simulink model "SWC_FDC_type"  (R2021b)
settings: Solver=FixedStepDiscrete  StartTime=0.0  StopTime=10.0  FixedStep=0.001  RelTol=1e-3
values from neighbouring files (symbols this model uses):
  C_TASK_5MS_S = (	C_TICK_TIME_S      	)    [vcu_local_hdr.m]
  DID_VCUKey = uint16(0x0202)    [vcu_local_hdr.m]
  DID_XWD = uint16(513)    [vcu_local_hdr.m]
  DIDLen_DKCKey = uint16(8)    [vcu_local_hdr.m]
  DIDLen_FoxPiBattSta = uint16(4)    [vcu_local_hdr.m]
  DIDLen_FoxPiBrakeSta = uint16(13)    [vcu_local_hdr.m]
  DIDLen_FoxPiButtonSta = uint16(2)    [vcu_local_hdr.m]
  DIDLen_FoxPiCtrlEnSw = uint16(1)    [vcu_local_hdr.m]
  DIDLen_FoxPiDrivingCtrl = uint16(21)    [vcu_local_hdr.m]
  DIDLen_FoxPiEPSSta = uint16(11)    [vcu_local_hdr.m]
  DIDLen_FoxPiLampCtrl = uint16(6)    [vcu_local_hdr.m]
  DIDLen_FoxPiLampSta = uint16(2)    [vcu_local_hdr.m]
  DIDLen_FoxPiMotionSta = uint16(13)    [vcu_local_hdr.m]
  DIDLen_FoxPiMotorSta = uint16(11)    [vcu_local_hdr.m]
  DIDLen_FoxPiPedalPos = uint16(3)    [vcu_local_hdr.m]
  DIDLen_FoxPiPTGUSSSw = uint16(1)    [vcu_local_hdr.m]
  DIDLen_FoxPiShifterAllow = uint16(3)    [vcu_local_hdr.m]
  DIDLen_FoxPiSwSta = uint16(2)    [vcu_local_hdr.m]
  DIDLen_FoxPiTPMSSta = uint16(13)    [vcu_local_hdr.m]
  DIDLen_FoxPiUSSDist = uint16(20)    [vcu_local_hdr.m]
  DIDLen_FoxPiUSSFaultSta = uint16(2)    [vcu_local_hdr.m]
  DIDLen_FoxPiWheelSpd = uint16(16)    [vcu_local_hdr.m]
  DIDNum_DKCKey = uint16(0x0202)    [vcu_local_hdr.m]
  DIDNum_FoxPiBattSta = uint16(0x100D)    [vcu_local_hdr.m]
  DIDNum_FoxPiBrakeSta = uint16(0x1003)    [vcu_local_hdr.m]
  DIDNum_FoxPiButtonSta = uint16(0x1006)    [vcu_local_hdr.m]
  DIDNum_FoxPiCtrlEnSw = uint16(0x1012)    [vcu_local_hdr.m]
  DIDNum_FoxPiDrivingCtrl = uint16(0x1001)    [vcu_local_hdr.m]
  DIDNum_FoxPiEPSSta = uint16(0x1005)    [vcu_local_hdr.m]
  DIDNum_FoxPiLampCtrl = uint16(0x100C)    [vcu_local_hdr.m]
  DIDNum_FoxPiLampSta = uint16(0x100B)    [vcu_local_hdr.m]
  DIDNum_FoxPiMotionSta = uint16(0x1002)    [vcu_local_hdr.m]
  DIDNum_FoxPiMotorSta = uint16(0x1010)    [vcu_local_hdr.m]
  DIDNum_FoxPiPedalPos = uint16(0x100F)    [vcu_local_hdr.m]
  DIDNum_FoxPiPTGUSSSw = uint16(0x1009)    [vcu_local_hdr.m]
  DIDNum_FoxPiShifterAllow = uint16(0x1011)    [vcu_local_hdr.m]
  DIDNum_FoxPiSwSta = uint16(0x100A)    [vcu_local_hdr.m]
  DIDNum_FoxPiTPMSSta = uint16(0x100E)    [vcu_local_hdr.m]
  DIDNum_FoxPiUSSDist = uint16(0x1007)    [vcu_local_hdr.m]
  DIDNum_FoxPiUSSFaultSta = uint16(0x1008)    [vcu_local_hdr.m]
  DIDNum_FoxPiWheelSpd = uint16(0x1004)    [vcu_local_hdr.m]
  DIDVCUKeyLength = uint16(8)    [vcu_local_hdr.m]
  DTC_10020B = Simulink.Parameter    [DTC_Constant_Definition.m]
  DTC_10020C = Simulink.Parameter    [DTC_Constant_Definition.m]
  DTC_10020D = Simulink.Parameter    [DTC_Constant_Definition.m]
  DTC_10020E = Simulink.Parameter    [DTC_Constant_Definition.m]
  DTC_100210 = Simulink.Parameter    [DTC_Constant_Definition.m]
  DTC_100211 = Simulink.Parameter    [DTC_Constant_Definition.m]
  DTC_100212 = Simulink.Parameter    [DTC_Constant_Definition.m]
  DTC_100213 = Simulink.Parameter    [DTC_Constant_Definition.m]
  DTC_100214 = Simulink.Parameter    [DTC_Constant_Definition.m]
  DTC_100215 = Simulink.Parameter    [DTC_Constant_Definition.m]
  DTC_100216 = Simulink.Parameter    [DTC_Constant_Definition.m]
  DTC_100217 = Simulink.Parameter    [DTC_Constant_Definition.m]
  DTC_100218 = Simulink.Parameter    [DTC_Constant_Definition.m]
  DTC_100219 = Simulink.Parameter    [DTC_Constant_Definition.m]
  DTC_10021A = Simulink.Parameter    [DTC_Constant_Definition.m]
  DTC_10021B = Simulink.Parameter    [DTC_Constant_Definition.m]
  DTC_10021C = Simulink.Parameter    [DTC_Constant_Definition.m]
  DTC_10021D = Simulink.Parameter    [DTC_Constant_Definition.m]
  DTC_10021E = Simulink.Parameter    [DTC_Constant_Definition.m]
  DTC_100220 = Simulink.Parameter    [DTC_Constant_Definition.m]
  DTC_100221 = Simulink.Parameter    [DTC_Constant_Definition.m]
  DTC_100223 = Simulink.Parameter    [DTC_Constant_Definition.m]
  DTC_100224 = Simulink.Parameter    [DTC_Constant_Definition.m]
  DTC_100225 = Simulink.Parameter    [DTC_Constant_Definition.m]
  DTC_100226 = Simulink.Parameter    [DTC_Constant_Definition.m]
  DTC_100227 = Simulink.Parameter    [DTC_Constant_Definition.m]
  DTC_100242 = Simulink.Parameter    [DTC_Constant_Definition.m]
  DTC_100243 = Simulink.Parameter    [DTC_Constant_Definition.m]
  DTC_100244 = Simulink.Parameter    [DTC_Constant_Definition.m]
  DTC_100247 = Simulink.Parameter    [DTC_Constant_Definition.m]
  DTC_100248 = Simulink.Parameter    [DTC_Constant_Definition.m]
  DTC_100249 = Simulink.Parameter    [DTC_Constant_Definition.m]
  DTC_100250 = Simulink.Parameter    [DTC_Constant_Definition.m]
  DTC_100251 = Simulink.Parameter    [DTC_Constant_Definition.m]
  DTC_100252 = Simulink.Parameter    [DTC_Constant_Definition.m]
  DTC_100A10 = Simulink.Parameter    [DTC_Constant_Definition.m]
  DTC_100A12 = Simulink.Parameter    [DTC_Constant_Definition.m]
  DTC_100A16 = Simulink.Parameter    [DTC_Constant_Definition.m]
  DTC_100A17 = Simulink.Parameter    [DTC_Constant_Definition.m]
  DTC_100A18 = Simulink.Parameter    [DTC_Constant_Definition.m]
  DTC_100A19 = Simulink.Parameter    [DTC_Constant_Definition.m]
  DTC_500B01 = Simulink.Parameter    [DTC_Constant_Definition.m]
  DTC_500B02 = Simulink.Parameter    [DTC_Constant_Definition.m]
  DTC_500B03 = Simulink.Parameter    [DTC_Constant_Definition.m]
  DTC_500B04 = Simulink.Parameter    [DTC_Constant_Definition.m]
  DTC_500B05 = Simulink.Parameter    [DTC_Constant_Definition.m]
  DTC_500B06 = Simulink.Parameter    [DTC_Constant_Definition.m]
  DTC_500B07 = Simulink.Parameter    [DTC_Constant_Definition.m]
  DTC_500B08 = Simulink.Parameter    [DTC_Constant_Definition.m]
  DTC_500B09 = Simulink.Parameter    [DTC_Constant_Definition.m]
  DTC_500B0A = Simulink.Parameter    [DTC_Constant_Definition.m]
  DTC_500B0B = Simulink.Parameter    [DTC_Constant_Definition.m]
  DTC_500B0C = Simulink.Parameter    [DTC_Constant_Definition.m]
  DTC_500B0D = Simulink.Parameter    [DTC_Constant_Definition.m]
  DTC_500B0E = Simulink.Parameter    [DTC_Constant_Definition.m]
  DTC_500B0F = Simulink.Parameter    [DTC_Constant_Definition.m]
  DTC_500B10 = Simulink.Parameter    [DTC_Constant_Definition.m]
  DTC_90021F = Simulink.Parameter    [DTC_Constant_Definition.m]
  DTC_90022F = Simulink.Parameter    [DTC_Constant_Definition.m]
  DTC_900253 = Simulink.Parameter    [DTC_Constant_Definition.m]
  DTC_900254 = Simulink.Parameter    [DTC_Constant_Definition.m]
  DTC_900301 = Simulink.Parameter    [DTC_Constant_Definition.m]
  DTC_900302 = Simulink.Parameter    [DTC_Constant_Definition.m]
  DTC_900303 = Simulink.Parameter    [DTC_Constant_Definition.m]
  DTC_900304 = Simulink.Parameter    [DTC_Constant_Definition.m]
  DTC_900305 = Simulink.Parameter    [DTC_Constant_Definition.m]
  DTC_900909 = Simulink.Parameter    [DTC_Constant_Definition.m]
  DTC_90090A = Simulink.Parameter    [DTC_Constant_Definition.m]
  DTC_90090B = Simulink.Parameter    [DTC_Constant_Definition.m]
  DTC_90090C = Simulink.Parameter    [DTC_Constant_Definition.m]
  DTC_90090D = Simulink.Parameter    [DTC_Constant_Definition.m]
  DTC_90090E = Simulink.Parameter    [DTC_Constant_Definition.m]
  DTC_90090F = Simulink.Parameter    [DTC_Constant_Definition.m]
  DTC_900910 = Simulink.Parameter    [DTC_Constant_Definition.m]
  DTC_900911 = Simulink.Parameter    [DTC_Constant_Definition.m]
  DTC_900912 = Simulink.Parameter    [DTC_Constant_Definition.m]
  DTC_900913 = Simulink.Parameter    [DTC_Constant_Definition.m]
  DTC_900914 = Simulink.Parameter    [DTC_Constant_Definition.m]
  ... (+54 more)
undefined symbols (not defined in the file or in its folder): f32_ApsOutVehSpdSig, KHAL_CANBusOffDebounce_cnt, KHAL_CANBusOffDebounce_s, KHAL_DKCDecryptEnable_flg_ovrdflg, KHAL_DKCDecryptEnable_flg_ovrdval, KHAL_RandomNumberY1_enum, KHAL_RandomNumberY2_enum, KHAL_RandomNumberY_ovrdflg, KHAL_TPMSRESBUTT_flg_ovrdflg, KHAL_TPMSRESBUTT_flg_ovrdval, KINP_ReadVinCode_flg, P_boolean, R_DIDWriteCDD_CSOP_DIDSet_DKCKey, R_DIDWriteCDD_CSOP_DIDSet_FoxPiBattSta, R_DIDWriteCDD_CSOP_DIDSet_FoxPiBrakeSta, R_DIDWriteCDD_CSOP_DIDSet_FoxPiButtonSta, R_DIDWriteCDD_CSOP_DIDSet_FoxPiCtrlEnSw, R_DIDWriteCDD_CSOP_DIDSet_FoxPiDrivingCtrl, R_DIDWriteCDD_CSOP_DIDSet_FoxPiEPSSta, R_DIDWriteCDD_CSOP_DIDSet_FoxPiLampCtrl, R_DIDWriteCDD_CSOP_DIDSet_FoxPiLampSta, R_DIDWriteCDD_CSOP_DIDSet_FoxPiMotionSta, R_DIDWriteCDD_CSOP_DIDSet_FoxPiMotorSta, R_DIDWriteCDD_CSOP_DIDSet_FoxPiPedalPos, R_DIDWriteCDD_CSOP_DIDSet_FoxPiPTGUSSSw, R_DIDWriteCDD_CSOP_DIDSet_FoxPiShifterAllow, R_DIDWriteCDD_CSOP_DIDSet_FoxPiSwSta, R_DIDWriteCDD_CSOP_DIDSet_FoxPiTPMSSta, R_DIDWriteCDD_CSOP_DIDSet_FoxPiUSSDist, R_DIDWriteCDD_CSOP_DIDSet_FoxPiUSSFaultSta, R_DIDWriteCDD_CSOP_DIDSet_FoxPiWheelSpd, R_E2E_CAN3_VCU1_CSOP_Write_CAN3_VCU1, R_E2E_CAN3_VCU1_toNIDEC_CSOP_Write_CAN3_VCU1_toNIDEC, R_E2E_CAN4_VCU1_CSOP_Write_CAN4_VCU1, R_FDCCDD_Inner_CSOP_FDC_AppCallSleep, R_HALIN_IMU_CSOP_IMUSetSta, R_HALINCDD_CSOP_PAS_Handler, R_HALINCDD_CSOP_ResetPedalZeroPosDone, R_HALINCDD_CSOP_TPMSSensorIDRegSetResults, R_HALINCDD_CSOP_UDS_Main, R_HALOUT_APS_CSOP_ApsOutput, R_HALOUTCDD_CSOP_AppNmStateReq, R_HALOUTCDD_CSOP_IVIReset, R_HALOUTCDD_CSOP_SetAcoreRebootCmdACK, R_HALOUTCDD_CSOP_SetSysPwrStat ... (+80)
libraries: FVT_lib x447, simulink x289, hcu_lib x19, hdlsllib x9, app x1, halin x1, halout x1, matrix_library x1, inp x1, outp x1
(part 3 of 15)

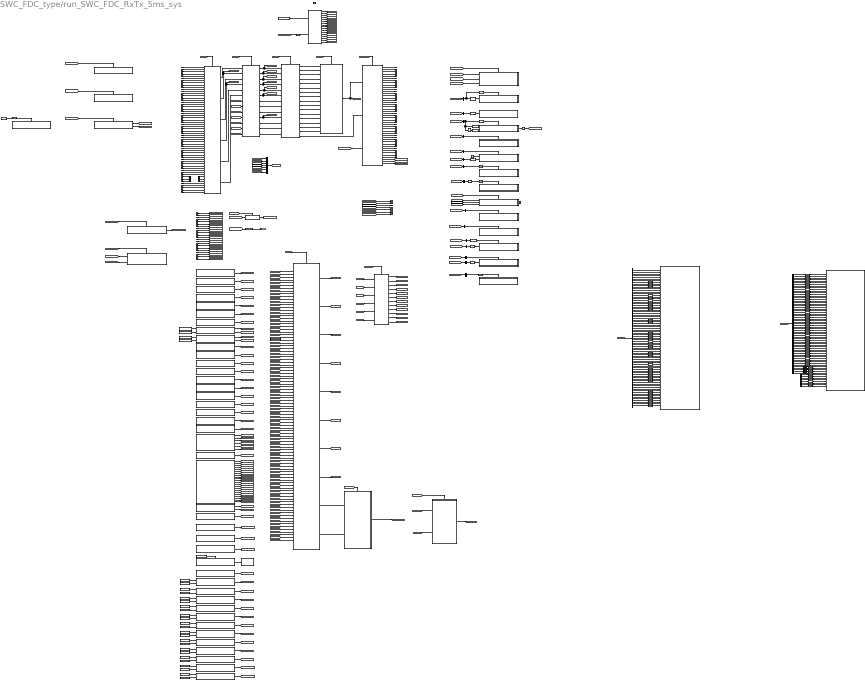
== system SWC_FDC_type/run_SWC_FDC_RxTx_5ms_sys ==
  R_CAN1_ABM1_CAN1_SG_ABM1_read : Inport
  R_CAN1_EPB1_CAN1_SG_EPB1_read : Inport  Port=2
  R_CAN1_EPS1_CAN1_SG_EPS1_read : Inport  Port=3
  R_CAN1_ESC1_CAN1_SG_ESC1_read : Inport  Port=4
  R_CAN1_ESC5_CAN1_SG_ESC5_read : Inport  Port=5
  R_CAN1_eBST1_CAN1_SG_eBST1_read : Inport  Port=6
  R_CAN2_HMI1_CAN2_SG_HMI1_read : Inport  Port=7
  R_CAN2_IVI1_CAN2_SG_IVI1_read : Inport  Port=8
  R_CAN2_IVI2_CAN2_SG_IVI2_read : Inport  Port=9
  R_CAN2_IVI3_CAN2_SG_IVI3_read : Inport  Port=10
  R_CAN2_METER1_CAN2_SG_METER1_read : Inport  Port=11
  R_CAN3_BMS1_CAN3_SG_BMS1_read : Inport  Port=12
  R_CAN3_BMS3_CAN3_SG_BMS3_read : Inport  Port=13
  R_CAN3_BMS4_CAN3_SG_BMS4_read : Inport  Port=14
  R_CAN3_BMS5_CAN3_SG_BMS5_read : Inport  Port=15
  R_CAN3_BMS6_CAN3_SG_BMS6_read : Inport  Port=16
  R_CAN3_BMS8_CAN3_SG_BMS8_read : Inport  Port=17
  R_CAN3_CCU1_CAN3_SG_CCU1_read : Inport  Port=18
  R_CAN3_CCU2_CAN3_SG_CCU2_read : Inport  Port=19
  R_CAN3_EBM1_CAN3_SG_EBM1_read : Inport  Port=20
  R_CAN3_MCU_B_F1_CAN3_SG_MCU_B_F1_read : Inport  Port=21
  R_CAN3_MCU_B_F2_CAN3_SG_MCU_B_F2_read : Inport  Port=22
  R_CAN3_MCU_B_R1_CAN3_SG_MCU_B_R1_read : Inport  Port=23
  R_CAN3_MCU_B_R2_CAN3_SG_MCU_B_R2_read : Inport  Port=24
  R_CAN3_MCU_N_F1_CAN3_SG_MCU_N_F1_read : Inport  Port=25
  R_CAN3_MCU_N_F2_CAN3_SG_MCU_N_F2_read : Inport  Port=26
  R_CAN3_MCU_N_F3_CAN3_SG_MCU_N_F3_read : Inport  Port=27
  R_CAN3_MCU_N_R1_CAN3_SG_MCU_N_R1_read : Inport  Port=28
  R_CAN3_MCU_N_R2_CAN3_SG_MCU_N_R2_read : Inport  Port=29
  R_CAN3_MCU_N_R3_CAN3_SG_MCU_N_R3_read : Inport  Port=30
  R_CAN3_Shifter1_CAN3_SG_Shifter1_read : Inport  Port=31
  R_CAN3_Shifter2_CAN3_SG_Shifter2_read : Inport  Port=32
  R_CAN4_BodyZone_DR1_CAN4_SG_BodyZone_DR1_read : Inport  Port=33
  R_CAN4_BodyZone_PS1_CAN4_SG_BodyZone_PS1_read : Inport  Port=34
  R_CAN4_BodyZone_PS2_CAN4_SG_BodyZone_PS2_read : Inport  Port=35
  R_CAN4_DKC1_CAN4_SG_DKC1_read : Inport  Port=36
  R_CAN4_DKC2_CAN4_SG_DKC2_read : Inport  Port=37
  R_CAN4_PTG1_CAN4_SG_PTG1_read : Inport  Port=38
  R_CAN4_ZONE_DR1_CAN4_SG_ZONE_DR1_read : Inport  Port=39
  R_CAN4_ZONE_DR_VCU_CAN4_SG_ZONE_DR_VCU_read : Inport  Port=40
  R_CAN4_ZONE_FR1_CAN4_SG_ZONE_FR1_read : Inport  Port=41
  R_CAN4_ZONE_FR_VCU_CAN4_SG_ZONE_FR_VCU_read : Inport  Port=42
  R_CAN4_zGW_APTC1_CAN4_SG_zGW_APTC1_read : Inport  Port=43
  R_CAN4_zGW_CANFr1_CAN4_SG_zGW_CANFr1_read : Inport  Port=44
  R_CAN4_zGW_LINDr1_CAN4_SG_zGW_LINDr1_read : Inport  Port=45
  R_CAN4_zGW_LINFr1_CAN4_SG_zGW_LINFr1_read : Inport  Port=46
  R_CAN4_zGW_SEAT1_CAN4_SG_zGW_SEAT1_read : Inport  Port=47
  R_CAN5_TBOX1_CAN5_SG_TBOX1_read : Inport  Port=48
  R_CAN5_TBOX2_CAN5_SG_TBOX2_read : Inport  Port=49
  R_CAN5_TBOX3_CAN5_SG_TBOX3_read : Inport  Port=50
  R_CAN6_FCM1_CAN6_SG_FCM1_read : Inport  Port=51
  R_CAN6_FCM3_CAN6_SG_FCM3_read : Inport  Port=52
  R_CAN6_FCM4_CAN6_SG_FCM4_read : Inport  Port=53
  R_CAN6_SRR1_CAN6_SG_SRR1_read : Inport  Port=54
  IRV_u16Array4_ApsInDist_read : Inport  Port=55
  IRV_u8Array12_ApsInUssSta_read : Inport  Port=56
  IRV_u8Array256_NvmReadArray_read : Inport  Port=57
  IRV_u8Array8_ApsInLevel_read : Inport  Port=58
  IRV_u8Array8_PasInDist_read : Inport  Port=59
  IRV_u8Array9_TPMSData_read : Inport  Port=60
  IRV_u8_ApsInPASChime_read : Inport  Port=61
  IRV_u8_ApsInSensorLayout_read : Inport  Port=62
  IRV_u8_ApsInSysFailSta_read : Inport  Port=63
  IRV_u8_ApsInSysMode_read : Inport  Port=64
  IRV_u8_CTDSW_read : Inport  Port=65
  IRV_u8_CrashSignal_read : Inport  Port=66
  IRV_u8_DrDoorSW_read : Inport  Port=67
  IRV_u8_HazardSW_read : Inport  Port=68
  IRV_u8_HoodSW_read : Inport  Port=69
  IRV_u8_PsDoorSW_read : Inport  Port=70
  IRV_u8_RLDoorSW_read : Inport  Port=71
  IRV_u8_RRDoorSW_read : Inport  Port=72
  IRV_u8_SeatSW_read : Inport  Port=73
  IRV_u8_TPMSDataInSta_read : Inport  Port=74
  IRV_u8_TailgateSW_read : Inport  Port=75
  IRV_u8_TrunkHanSW_read : Inport  Port=76
  R_CAN4_zGW_LINDr2_CAN4_SG_zGW_LINDr2_read : Inport  Port=77
  R_CAN4_zGW_LINFr2_CAN4_SG_zGW_LINFr2_read : Inport  Port=78
  R_CAN6_FCM2_CAN6_SG_FCM2_read : Inport  Port=79
  R_CAN4_BodyZone_DR2_CAN4_SG_BodyZone_DR2_read : Inport  Port=80
  function : TriggerPort  TriggerType=function-call  VariantControl=(inherit)  SampleTimeType=periodic  SampleTime=-1
  APP : app/APP  SystemSampleTime=-1  VariantActivationTime=update diagram  Latency=0  AutoFrameSizeCalculation=off
  Bus Creator : BusCreator  Inputs=7
  Bus Selector : BusSelector  OutputSignals=VOUTP_EnterNewOperCyc_flg
  Bus Selector1 : BusSelector  OutputSignals=VOUTP_AcoreRebootCmdACK_flg
  Bus Selector10 : BusSelector  OutputSignals=VOUTP_NetworkReq_flg
  Bus Selector11 : BusSelector  OutputSignals=VOUTP_SysPowerMode_enum
  Bus Selector12 : BusSelector  OutputSignals=VOUTP_NvWriteReqRisingEdge_flg
  Bus Selector13 : BusSelector  OutputSignals=VOUTP_FdcSlpReqRisingEdge_flg
  Bus Selector14 : BusSelector  OutputSignals=VOUTP_FdcSlpReqRisingEdge_flg
  Bus Selector15 : BusSelector  OutputSignals=VOUTP_FdcSlpReqRisingEdge_flg
  Bus Selector16 : BusSelector  OutputSignals=VOUTP_FdcSlpTime_sec
  Bus Selector17 : BusSelector  OutputSignals=VOUTP_IVIRST_flg
  Bus Selector2 : BusSelector  OutputSignals=VOUTP_IMUEnaCmd_flg
  Bus Selector3 : BusSelector  OutputSignals=VOUTP_PowerSta_enum,VOUTP_BrkPedalPos_pct,VOUTP_ActAPSPosn_pct,VOUTP_LFRawWhlSpeed_kph,VOUTP_RFRawWhlSpeed_kph,VOUTP_LRRawWhlSpeed_kph,VOUTP_RRRawWhlSpeed_kph,VOUTP_LFRawWhlSpeedV_flg,VOUTP_RFRawWhlSpeedV_flg,VOUTP_LRRawWhlSpeedV_flg,VOUTP_RRRawWhlSpeedV_flg,VOUTP_LFWhlRotDir_enum,VOUTP_RFWhlRotDir_enum,VOUTP_LRWhlRotDir_enum,VOUTP_RRWhlRotDir_enum,VOUTP_LFPulseCountV_flg,VOUTP_RFPulseCountV_flg,VOUTP_LRPulseCountV_flg,VOUTP_RRPulseCountV_flg,VOUTP_LFPulseCount_enum,VOUTP_RFPulseCount_enum,VOUTP_LRPulseCount_enum,VOUTP_RRPulseCount_enum,VOUTP_APSActive_flg,VOUTP_APSCtrlAvail_flg,VOUTP_ShifterHandleCmd_enum,VOUTP_DriIntend_enum,VOUTP_EPSAOIControl_enum,VOUTP_SASAngle_Deg,VOUTP_SASSpeed_degps,VOUTP_SASSpeedValid_flg,VOUTP_SASCAL_flg,VOUTP_SASV_flg,VOUTP_GRADE_Deg,VOUTP_YawRate_degps,VOUTP_LatAccel_Gps,VOUTP_LongAccel_Gps,VOUTP_MCPressure_bar,VOUTP_YawRateV_flg,VOUTP_LatAccelV_flg,VOUTP_LongAccelV_flg,VOUTP_MCPressureV_bar,VOUTP_BrkSwSta_flg,VOUTP_BrkSwV_flg,VOUTP_ESCStandstill_flg,VOUTP_ESCAPSSta_enum,VOUTP_EPBExtReleaseAvail_flg,VOUTP_EPBExtApplyAvail_flg,VOUTP_EPBErrSta_enum,VOUTP_EPBSta_enum,VOUTP_AllDoorSW_flg,VOUTP_HoodSW_flg,VOUTP_TailgateSW_flg,VOUTP_AVMparkingcancel_enum,VOUTP_AVMparkingexcute_enum,VOUTP_AVMParkingmode_enum,VOUTP_AVMErrSTA_flg,VOUTP_IVIStatus_flg,VOUTP_CAASSw_enum,VOUTP_IVIScreen_enum,VOUTP_CAASCtrlAvail_flg,VOUTP_ABSActive_flg,VOUTP_TCSActive_flg,VOUTP_DriverSeatBeltCmd_flg,VOUTP_DrDoorSW_flg,VOUTP_PsDoorSW_flg,VOUTP_RLDoorSW_flg,VOUTP_RRDoorSW_flg,VOUTP_RFPressIndi_enum,VOUTP_LFPressIndi_enum,VOUTP_RRPressIndi_enum,VOUTP_LRPressIndi_enum,VOUTP_sigAmbAirT_C,VOUTP_VehActSpd_kph,VOUTP_CAASActive_flg,VOUTP_PwrReqRAPSAvail_flg,VOUTP_DKCPDkeyAreaRAPSSta_enum,VOUTP_DKCParkingModeCmd_enum,VOUTP_PUIDLowPower_flg,VOUTP_DrSeatSta_enum,VOUTP_VCURAPSErrLv2_flg,VOUTP_VCURAPSErrLv3_flg,VOUTP_IVIUserTakeOverAPSSta_flg
  Bus Selector4 : BusSelector  OutputSignals=VOUTP_BrkPedalPosTimeOut_flg,VOUTP_LFRawWhlSpeedTimeOut_flg,VOUTP_RFRawWhlSpeedTimeOut_flg,VOUTP_LRRawWhlSpeedTimeOut_flg,VOUTP_RRRawWhlSpeedTimeOut_flg,VOUTP_LFRawWhlSpeedVTimeOut_flg,VOUTP_RFRawWhlSpeedVTimeOut_flg,VOUTP_LRRawWhlSpeedVTimeOut_flg,VOUTP_RRRawWhlSpeedVTimeOut_flg,VOUTP_LFWhlRotDirTimeOut_flg,VOUTP_RFWhlRotDirTimeOut_flg,VOUTP_LRWhlRotDirTimeOut_flg,VOUTP_RRWhlRotDirTimeOut_flg,VOUTP_LFPulseCountVTimeOut_flg,VOUTP_RFPulseCountVTimeOut_flg,VOUTP_LRPulseCountVTimeOut_flg,VOUTP_RRPulseCountVTimeOut_flg,VOUTP_LFPulseCountTimeOut_flg,VOUTP_RFPulseCountTimeOut_flg,VOUTP_LRPulseCountTimeOut_flg,VOUTP_RRPulseCountTimeOut_flg,VOUTP_ShifterHandleCmdTimeOut_flg,VOUTP_DriIntendTimeOut_flg,VOUTP_EPSAOIControlTimeOut_flg,VOUTP_SASAngleTimeOut_flg,VOUTP_SASSpeedTimeOut_flg,VOUTP_SASSpeedValidTimeOut_flg,VOUTP_SASCALTimeOut_flg,VOUTP_SASVTimeOut_flg,VOUTP_GRADETimeOut_flg,VOUTP_YawRateTimeOut_flg,VOUTP_LatAccelTimeOut_flg,VOUTP_LongAccelTimeOut_flg,VOUTP_MCPressureTimeOut_flg,VOUTP_YawRateVTimeOut_flg,VOUTP_LatAccelVTimeOut_flg,VOUTP_LongAccelVTimeOut_flg,VOUTP_MCPressureVTimeOut_flg,VOUTP_BrkSwStaTimeOut_flg,VOUTP_BrkSwVTimeOut_flg,VOUTP_ESCStandstillTimeOut_flg,VOUTP_ESCAPSStaTimeOut_flg,VOUTP_EPBExtReleaseAvailTimeOut_flg,VOUTP_EPBExtApplyAvailTimeOut_flg,VOUTP_EPBErrStaTimeOut_flg,VOUTP_EPBStaTimeOut_flg,VOUTP_AVMparkingcancelTimeOut_flg,VOUTP_AVMparkingexcuteTimeOut_flg,VOUTP_AVMParkingmodeTimeOut_flg,VOUTP_AVMErrSTATimeOut_flg,VOUTP_IVIStatusTimeOut_flg,VOUTP_CAASSwTimeOut_flg,VOUTP_IVIScreenTimeOut_flg,VOUTP_ABSActiveTimeOut_flg,VOUTP_TCSActiveTimeOut_flg,VOUTP_DriverSeatBeltCmdTimeOut_flg,VOUTP_RFPressIndi_enum,VOUTP_LFPressIndi_enum,VOUTP_RRPressIndi_enum,VOUTP_LRPressIndi_enum,VOUTP_sigAmbAirT_C
  Bus Selector5 : BusSelector  OutputSignals=VOUTP_IMUEnaCmd_flg
  Bus Selector6 : BusSelector  OutputSignals=VHAL_TPMSSensorIDRegResults_raw8
  Bus Selector7 : BusSelector  OutputSignals=VOUTP_TPMSSensorIDRegStart_flg
  Bus Selector8 : BusSelector  OutputSignals=VOUTP_ResetPedalZeroPosStart_flg
  Constant : Constant  Value=DIDVCUKeyLength
  Constant1 : Constant  Value=DID_VCUKey
  Constant{7,10,16..17,21,25,29} (7 alike) : Constant  Value=ZERO_INT
  Constant{6,9,11..13,20,24,28,32} (9 alike) : Constant  Value=ONE_INT
  Constant14 : Constant  Value=TWO_INT
  Constant15 : Constant  Value=TWO_INT
  Constant18 : Constant  Value=THREE_INT
  Constant19 : Constant  Value=THREE_INT
  Constant2 : Constant  Value=uint16(ONE_INT)
  Constant22 : Constant  Value=FOUR_INT
  Constant23 : Constant  Value=FOUR_INT
  Constant26 : Constant  Value=FIVE_INT
  Constant27 : Constant  Value=FIVE_INT
  Constant3 : Constant  Value=DID_XWD
  Constant30 : Constant  Value=SIX_INT
  Constant31 : Constant  Value=SIX_INT
  Constant4 : Constant  Value=TRUE
  Constant5 : Constant  Value=FALSE
  Constant8 : Constant  Value=KINP_ReadVinCode_flg
  DIDGet_Subsystem : Subsystem
  DIDSet_Subsystem : Subsystem
  Data Type Conversion{,1..3,5..13,17..19,21..95,97..107,109..125} (119 alike) : DataTypeConversion  OutDataTypeStr=uint8
  Data Type Conversion{14..16,20} (4 alike) : DataTypeConversion  OutDataTypeStr=int16
  Data Type Conversion4 : DataTypeConversion  OutDataTypeStr=uint32
  Data Type Conversion96 : DataTypeConversion  OutDataTypeStr=single
  Detect Increase : simulink/Logic and Bit Operations/Detect Increase  vinit=0.0  OutDataTypeStr=boolean
  Detect Increase1 : simulink/Logic and Bit Operations/Detect Increase  vinit=0.0  OutDataTypeStr=boolean
  Display : Display
  Function-Call Subsystem : Subsystem  TreatAsAtomicUnit=on
  Ground{,1..8} (9 alike) : Ground
  Ground_{18..24,26} (8 alike) : Ground
  HALOUT_AFTER : Subsystem
  HAL_IN : halin/HAL_IN  SystemSampleTime=-1  VariantActivationTime=update diagram  Latency=0  AutoFrameSizeCalculation=off
  HAL_OUT : halout/HAL_OUT  SystemSampleTime=-1  VariantActivationTime=update diagram  Latency=0  AutoFrameSizeCalculation=off
  Halin_CDD : Subsystem
      settings: RTWSystemCode=Nonreusable function  RTWFcnNameOpts=Use subsystem name  RTWFileNameOpts=Use subsystem name
  INP : inp/INP  SystemSampleTime=-1  VariantActivationTime=update diagram  Latency=0  AutoFrameSizeCalculation=off
  Latch : hcu_lib/Basic_Blocks/Latch
  NOT : Logic  Operator=NOT  Inputs=1  AllPortsSameDT=off  OutDataTypeStr=boolean
  OUTP : outp/OUTP  SystemSampleTime=-1  VariantActivationTime=update diagram  Latency=0  AutoFrameSizeCalculation=off
  OUTP_AFTER : Subsystem
      settings: RTWSystemCode=Nonreusable function  RTWFcnNameOpts=Use subsystem name  RTWFileNameOpts=Use subsystem name
  R_FDCCDD_Inner_CSOP_FDC_AppCallSleep : Subsystem
  R_HALINCDD_CSOP_AnyNmID : FunctionCaller  FunctionPrototype=u8_AnyNMID = R_HALINCDD_CSOP_AnyNmID()  OutputArgumentSpecifications=uint8(1)
  R_HALINCDD_CSOP_CAN1BusOff : FunctionCaller  FunctionPrototype=u8_CAN1BusOff = R_HALINCDD_CSOP_CAN1BusOff()  OutputArgumentSpecifications=uint8(1)
  R_HALINCDD_CSOP_CAN2BusOff : FunctionCaller  FunctionPrototype=u8_CAN2BusOff = R_HALINCDD_CSOP_CAN2BusOff()  OutputArgumentSpecifications=uint8(1)
  R_HALINCDD_CSOP_CAN3BusOff : FunctionCaller  FunctionPrototype=u8_CAN3BusOff = R_HALINCDD_CSOP_CAN3BusOff()  OutputArgumentSpecifications=uint8(1)
  R_HALINCDD_CSOP_CAN4BusOff : FunctionCaller  FunctionPrototype=u8_CAN4BusOff = R_HALINCDD_CSOP_CAN4BusOff()  OutputArgumentSpecifications=uint8(1)
  R_HALINCDD_CSOP_CAN5BusOff : FunctionCaller  FunctionPrototype=u8_CAN5BusOff = R_HALINCDD_CSOP_CAN5BusOff()  OutputArgumentSpecifications=uint8(1)
  R_HALINCDD_CSOP_CAN6BusOff : FunctionCaller  FunctionPrototype=u8_CAN6BusOff = R_HALINCDD_CSOP_CAN6BusOff()  OutputArgumentSpecifications=uint8(1)
  R_HALINCDD_CSOP_DIDgetDKCdata : FunctionCaller  FunctionPrototype=[u8_DidStaDKC,u8Array8_DidDataDKC] = R_HALINCDD_CSOP_DIDgetDKCdata(u16_lengthDIDDKC,u16_DIDDKC)  InputArgumentSpecifications=uint16(1), uint16(1)  OutputArgumentSpecifications=uint8(1), uint8([1;1;1;1;1;1;1;1])
  R_HALINCDD_CSOP_DIDgetXWDdata : FunctionCaller  FunctionPrototype=[u8_DidStaXWD,u8_DidDataXWD] = R_HALINCDD_CSOP_DIDgetXWDdata(u16_lengthDIDXWD,u16_DIDXWD)  InputArgumentSpecifications=uint16(1), uint16(1)  OutputArgumentSpecifications=uint8(1), uint8(1)
  R_HALINCDD_CSOP_GetAcoreReadyToSleep : FunctionCaller  FunctionPrototype=s8_AcoreReadyToSleep = R_HALINCDD_CSOP_GetAcoreReadyToSleep()  OutputArgumentSpecifications=int8(1)
  R_HALINCDD_CSOP_GetAcoreRebootCmd : FunctionCaller  FunctionPrototype=u8_AcoreRebootCmd = R_HALINCDD_CSOP_GetAcoreRebootCmd()  OutputArgumentSpecifications=uint8(1)
  R_HALINCDD_CSOP_GetAuxBattVoltage : FunctionCaller  FunctionPrototype=u16_AuxBattVol100mV = R_HALINCDD_CSOP_GetAuxBattVoltage()  OutputArgumentSpecifications=uint16(1)
  R_HALINCDD_CSOP_GetBootPath : FunctionCaller  FunctionPrototype=u32_BootPath = R_HALINCDD_CSOP_GetBootPath()  OutputArgumentSpecifications=uint32(1)
  R_HALINCDD_CSOP_GetBootReason : FunctionCaller  FunctionPrototype=u8_BootReason = R_HALINCDD_CSOP_GetBootReason()  OutputArgumentSpecifications=uint8(1)
  R_HALINCDD_CSOP_GetEvccAplusPwrUpReq : FunctionCaller  FunctionPrototype=u8_EvccAplusPwrUpReq = R_HALINCDD_CSOP_GetEvccAplusPwrUpReq()  OutputArgumentSpecifications=uint8(1)
  R_HALINCDD_CSOP_GetNmState : FunctionCaller  FunctionPrototype=u8_CurrentNMState = R_HALINCDD_CSOP_GetNmState()  OutputArgumentSpecifications=uint8(1)
  R_HALINCDD_CSOP_GetNvmProtectState : FunctionCaller  FunctionPrototype=u8_NvmProtectSta = R_HALINCDD_CSOP_GetNvmProtectState()  OutputArgumentSpecifications=uint8(1)
  R_HALINCDD_CSOP_GetSWID : FunctionCaller  FunctionPrototype=u8Array33_SWID = R_HALINCDD_CSOP_GetSWID()  OutputArgumentSpecifications=uint8([1;1;1;1;1;1;1;1;1;1;1;1;1;1;1;1;1;1;1;1;1;1;1;1;1;1;1;1;1;1;1;1;1])
  R_HALINCDD_CSOP_GetVinpAllowMoveThdOta : FunctionCaller  FunctionPrototype=u8_AllowMovThdOTA = R_HALINCDD_CSOP_GetVinpAllowMoveThdOta()  OutputArgumentSpecifications=uint8(1)
  R_HALINCDD_CSOP_GetVinpPwrReqOta : FunctionCaller  FunctionPrototype=u8_PwrReqOTA = R_HALINCDD_CSOP_GetVinpPwrReqOta()  OutputArgumentSpecifications=uint8(1)
  R_HALINCDD_CSOP_GetWISR : FunctionCaller  FunctionPrototype=u32_WISR = R_HALINCDD_CSOP_GetWISR()  OutputArgumentSpecifications=uint32(1)
  R_HALINCDD_CSOP_HALINCDD_DIRECT : FunctionCaller  FunctionPrototype=[u8_BrakeSW,u8_BrakeLamp,u16_Pedal1Vol,u16_Pedal2Vol,u16_Pedal1Ref5V,u16_Pedal2Ref5V] = R_HALINCDD_CSOP_HALINCDD_DIRECT()  OutputArgumentSpecifications=uint8(1), uint8(1), uint16(1), uint16(1), uint16(1), uint16(1)
  R_HALINCDD_CSOP_ReadPedalZeroPosReq : FunctionCaller  FunctionPrototype=u8_ReadPedalZeroPosReq = R_HALINCDD_CSOP_ReadPedalZeroPosReq()  OutputArgumentSpecifications=uint8(1)
  R_HALINCDD_CSOP_ResetPedalZeroPosReq : FunctionCaller  FunctionPrototype=u8_ResetPedalZeroPosReq = R_HALINCDD_CSOP_ResetPedalZeroPosReq()  OutputArgumentSpecifications=uint8(1)
  R_HALINCDD_CSOP_TPMSSensorIDRegGetSta : FunctionCaller  FunctionPrototype=u8_TPMSSensorIDRegSta = R_HALINCDD_CSOP_TPMSSensorIDRegGetSta()  OutputArgumentSpecifications=uint8(1)
  R_HALINCDD_CSOP_nmGetCan1RxErrorCount : FunctionCaller  FunctionPrototype=u8_pCan1RxErrorCount = R_HALINCDD_CSOP_nmGetCan1RxErrorCount(u8_canChannel,u8_isGetRx)  InputArgumentSpecifications=uint8(1), uint8(1)  OutputArgumentSpecifications=uint8(1)
  R_HALINCDD_CSOP_nmGetCan1TxErrorCount : FunctionCaller  FunctionPrototype=u8_pCan1TxErrorCount = R_HALINCDD_CSOP_nmGetCan1TxErrorCount(u8_canChannel,u8_isGetRx)  InputArgumentSpecifications=uint8(1), uint8(1)  OutputArgumentSpecifications=uint8(1)
  R_HALINCDD_CSOP_nmGetCan2RxErrorCount : FunctionCaller  FunctionPrototype=u8_pCan2RxErrorCount = R_HALINCDD_CSOP_nmGetCan2RxErrorCount(u8_canChannel,u8_isGetRx)  InputArgumentSpecifications=uint8(1), uint8(1)  OutputArgumentSpecifications=uint8(1)
  R_HALINCDD_CSOP_nmGetCan2TxErrorCount : FunctionCaller  FunctionPrototype=u8_pCan2TxErrorCount = R_HALINCDD_CSOP_nmGetCan2TxErrorCount(u8_canChannel,u8_isGetRx)  InputArgumentSpecifications=uint8(1), uint8(1)  OutputArgumentSpecifications=uint8(1)
  R_HALINCDD_CSOP_nmGetCan3RxErrorCount : FunctionCaller  FunctionPrototype=u8_pCan3RxErrorCount = R_HALINCDD_CSOP_nmGetCan3RxErrorCount(u8_canChannel,u8_isGetRx)  InputArgumentSpecifications=uint8(1), uint8(1)  OutputArgumentSpecifications=uint8(1)
  R_HALINCDD_CSOP_nmGetCan3TxErrorCount : FunctionCaller  FunctionPrototype=u8_pCan3TxErrorCount = R_HALINCDD_CSOP_nmGetCan3TxErrorCount(u8_canChannel,u8_isGetRx)  InputArgumentSpecifications=uint8(1), uint8(1)  OutputArgumentSpecifications=uint8(1)
  R_HALINCDD_CSOP_nmGetCan4RxErrorCount : FunctionCaller  FunctionPrototype=u8_pCan4RxErrorCount = R_HALINCDD_CSOP_nmGetCan4RxErrorCount(u8_canChannel,u8_isGetRx)  InputArgumentSpecifications=uint8(1), uint8(1)  OutputArgumentSpecifications=uint8(1)
  R_HALINCDD_CSOP_nmGetCan4TxErrorCount : FunctionCaller  FunctionPrototype=u8_pCan4TxErrorCount = R_HALINCDD_CSOP_nmGetCan4TxErrorCount(u8_canChannel,u8_isGetRx)  InputArgumentSpecifications=uint8(1), uint8(1)  OutputArgumentSpecifications=uint8(1)
  R_HALINCDD_CSOP_nmGetCan5RxErrorCount : FunctionCaller  FunctionPrototype=u8_pCan5RxErrorCount = R_HALINCDD_CSOP_nmGetCan5RxErrorCount(u8_canChannel,u8_isGetRx)  InputArgumentSpecifications=uint8(1), uint8(1)  OutputArgumentSpecifications=uint8(1)
  R_HALINCDD_CSOP_nmGetCan5TxErrorCount : FunctionCaller  FunctionPrototype=u8_pCan5TxErrorCount = R_HALINCDD_CSOP_nmGetCan5TxErrorCount(u8_canChannel,u8_isGetRx)  InputArgumentSpecifications=uint8(1), uint8(1)  OutputArgumentSpecifications=uint8(1)
  R_HALINCDD_CSOP_nmGetCan6RxErrorCount : FunctionCaller  FunctionPrototype=u8_pCan6RxErrorCount = R_HALINCDD_CSOP_nmGetCan6RxErrorCount(u8_canChannel,u8_isGetRx)  InputArgumentSpecifications=uint8(1), uint8(1)  OutputArgumentSpecifications=uint8(1)
  R_HALINCDD_CSOP_nmGetCan6TxErrorCount : FunctionCaller  FunctionPrototype=u8_pCan6TxErrorCount = R_HALINCDD_CSOP_nmGetCan6TxErrorCount(u8_canChannel,u8_isGetRx)  InputArgumentSpecifications=uint8(1), uint8(1)  OutputArgumentSpecifications=uint8(1)
  R_HALINCDD_u8Array4_HWID : FunctionCaller  FunctionPrototype=u8Array4_HWID = R_HALINCDD_u8Array4_HWID()  OutputArgumentSpecifications=uint8([1;1;1;1])
  R_HALIN_APS_CSOP_ApsGetData : FunctionCaller  FunctionPrototype=[u8_GetAPS_Progress_PCT,u8_GetAPS_RQ_Display,u8_GetAPS_SW_Ver,u8_GetAPS_HW_Ver,u8_GetAPS_ExitCondition,f32_GetAPS_Angle_Target,u8_GetAPS_Sta_System,u8_GetAPS_V_Rq_EPAS_Ctrl,u8_GetAPS_Rq_EPAS_Ctrl,u8_GetAPS_Req,f32_GetAPS_DecReq,u8_GetAPS_DecReq_A,f32_GetAPS_SpeedCmd,u8_GetAPS_ShftPosnReq,u8_GetAPS_VMC_Req_A,u8_GetCAAS_Sta,u8_GetCAAS_VMC_Req_A,u8_GetAPS_PwrReq_cmd,u8_GetRAPS_BCM_LockReq_Cmd,u8_GetRAPS_BCM_Lamp_Cmd,u8_GetRAPS_ErrWarn_Sta,u8_GetRAPS_ErrLv1_flg] = R_HALIN_APS_CSOP_ApsGetData()  OutputArgumentSpecifications=uint8(1), uint8(1), uint8(1), uint8(1), uint8(1), single(1), uint8(1), uint8(1), uint8(1), uint8(1), single(1), uint8(1), single(1), uint8(1), uint8(1), uint8(1), uint8(1), uint8(1), uint8(1), uint8(1), uint8(1), uint8(1)
  R_HALIN_IMU_CSOP_IMUGetOffsetVal : Subsystem
  R_HALIN_IMU_CSOP_IMUGetSixAxisVal : FunctionCaller  FunctionPrototype=[s16_IMUSixAxisVal,u8_IMUSixAxisValSta] = R_HALIN_IMU_CSOP_IMUGetSixAxisVal()  OutputArgumentSpecifications=int16([1;1;1;1;1;1]), uint8(1)
  R_HALIN_IMU_CSOP_IMUSetSta : Subsystem
  R_HALOUTCDD_CSOP_AppNmStateReq : Subsystem
  R_HALOUTCDD_CSOP_SetAcoreRebootCmdACK : Subsystem
  R_HALOUTCDD_CSOP_SetSysPwrStat : FunctionCaller  FunctionPrototype=R_HALOUTCDD_CSOP_SetSysPwrStat(u8_SysPwrStat)  InputArgumentSpecifications=uint8(1)
  R_HALOUTCDD_CSOP_SleepRequest : Subsystem
  R_HALOUT_APS_CSOP_ApsSetData : FunctionCaller  FunctionPrototype=R_HALOUT_APS_CSOP_ApsSetData(u8_SetPwrSta,f32_SetBrkPedalPos,f32_SetActAPSPosn,f32_SetLF_RawWhlSpeed,f32_SetRF_RawWhlSpeed,f32_SetLR_RawWhlSpeed,f32_SetRR_RawWhlSpeed,u8_SetLF_RawWhlSpeed_V,u8_SetRF_RawWhlSpeed_V,u8_SetLR_RawWhlSpeed_V,u8_SetRR_RawWhlSpeed_V,u8_SetLF_WhlRotDir,u8_SetRF_WhlRotDir,u8_SetLR_WhlRotDir,u8_SetRR_WhlRotDir,u8_SetLF_PulseCount_V,u8_SetRF_PulseCount_V,u8_SetLR_PulseCount_V,u8_SetRR_PulseCount_V,s16_SetLF_PulseCount,s16_SetRF_PulseCount,s16_SetLR_PulseCount,s16_SetRR_PulseCount,u8_SetAPS_Active,u8_SetAPS_CtrlAvail,u8_SetShifter_Handle_Cmd,u8_SetDriIntend,u8_SetEPS_AOI_Control,f32_SetSAS_Angle,f32_SetSAS_Speed,u8_SetSAS_Speed_Valid,u8_SetSAS_CAL,u8_SetSAS_OK,f32_SetGRADE,f32_SetYawRate,f32_SetLatAccel,f32_SetLongAccel,f32_SetMCPressure,u8_SetYawRate_V,u8_SetLatAccel_V,u8_SetLongAccel_V,u8_SetMCPressure_V,u8_SetBrkSw_Sta,u8_SetBrkSw_V,u8_SetESC_Standstill,u8_SetESC_APS_Sta,u8_SetEPBExtReleaseAvail,u8_SetEPBExtApplyAvail,u8_SetEPBErrSta,u8_SetEPBSta,u8_SetAllDoorSW,u8_SetHoodSW,u8_SetTailgate_SW,u8_SetAVM_parking_cancel,u8_SetAVM_parking_excute,u8_SetAVM_Parking_mode,u8_SetAVM_Err_STA,u8_SetIVI_Status,u8_SetCAAS_Sw,u8_SetIVI_Screen,u8_SetCAAS_CtrlAvail,u8_SetABS_Active,u8_SetTCS_Active,u8_SetDriverSeatBeltCmd,u8_SetDrDoorSW,u8_SetPsDoorSW,u8_SetRLDoorSW,u8_SetRRDoorSW,u8_SetRFPressIndi,u8_SetLFPressIndi,u8_SetRRPressIndi,u8_SetLRPressIndi,f32_SetsigAmbAirT,f32_SetVehActSpd,u8_SetCAAS_Active,u8_SetAPS_PwrReqAvail_sta,u8_SetDKC_PDkeyAreaRAPS_Sta,u8_SetDKC_ParkingMode_Cmd,u8_SetP_UID_LowPower,u8_SetDr_SeatSta,u8_SetVCU_RAPSErrLv2_flg,u8_SetVCU_RAPSErrLv3_flg,u8_SetIVI_UserTakeOver_APS_Sta)  InputArgumentSpecifications=uint8(1), single(1), single(1), single(1), single(1), single(1), single(1), uint8(1), uint8(1), uint8(1), uint8(1), uint8(1), uint8(1), uint8(1), uint8(1), uint8(1), uint8(1), uint8(1), uint8(1), int16(1), int16(1), int16(1), int16(1), uint8(1), uint8(1), uint8(1), uint8(1), uint8(1), single(1), single(1), uint8(1), uint8(1), uint8(1), single(1), single(1), single(1), single(1), single(1), uint8(1), uint8(1), uint8(1), uint8(1), uint8(1), uint8(1), uint8(1), uint8(1), uint8(1), uint8(1), uint8(1), uint8(1), uint8(1), uint8(1), uint8(1), uint8(1), uint8(1), uint8(1), uint8(1), uint8(1), uint8(1), uint8(1), uint8(1), uint8(1), uint8(1), uint8(1), uint8(1), uint8(1), uint8(1), uint8(1), uint8(1), uint8(1), uint8(1), uint8(1), single(1), single(1), uint8(1), uint8(1), uint8(1), uint8(1), uint8(1), uint8(1), uint8(1), uint8(1), uint8(1)
  R_HALOUT_APS_CSOP_ApsSetTimeout : FunctionCaller  FunctionPrototype=R_HALOUT_APS_CSOP_ApsSetTimeout(u8_SetBrkPedalPosTO,u8_SetLF_RawWhlSpeedTO,u8_SetRF_RawWhlSpeedTO,u8_SetLR_RawWhlSpeedTO,u8_SetRR_RawWhlSpeedTO,u8_SetLF_RawWhlSpeed_VTO,u8_SetRF_RawWhlSpeed_VTO,u8_SetLR_RawWhlSpeed_VTO,u8_SetRR_RawWhlSpeed_VTO,u8_SetLF_WhlRotDirTO,u8_SetRF_WhlRotDirTO,u8_SetLR_WhlRotDirTO,u8_SetRR_WhlRotDirTO,u8_SetLF_PulseCount_VTO,u8_SetRF_PulseCount_VTO,u8_SetLR_PulseCount_VTO,u8_SetRR_PulseCount_VTO,u8_SetLF_PulseCountTO,u8_SetRF_PulseCountTO,u8_SetLR_PulseCountTO,u8_SetRR_PulseCountTO,u8_SetShifter_Handle_CmdTO,u8_SetDriIntendTO,u8_SetEPS_AOI_ControlTO,u8_SetSAS_AngleTO,u8_SetSAS_SpeedTO,u8_SetSAS_Speed_ValidTO,u8_SetSAS_CALTO,u8_SetSAS_OKTO,u8_SetGRADETO,u8_SetYawRateTO,u8_SetLatAccelTO,u8_SetLongAccelTO,u8_SetMCPressureTO,u8_SetYawRate_VTO,u8_SetLatAccel_VTO,u8_SetLongAccel_VTO,u8_SetMCPressure_VTO,u8_SetBrkSw_StaTO,u8_SetBrkSw_VTO,u8_SetESC_StandstillTO,u8_SetESC_APS_StaTO,u8_SetEPBExtReleaseAvailTO,u8_SetEPBExtApplyAvailTO,u8_SetEPBErrStaTO,u8_SetEPBStaTO,u8_SetAVM_parking_cancelTO,u8_SetAVM_parking_excuteTO,u8_SetAVM_Parking_modeTO,u8_SetAVM_Err_STATO,u8_SetIVI_StatusTO,u8_SetCAAS_SwTO,u8_SetIVI_ScreenTO,u8_SetABS_ActiveTO,u8_SetTCS_ActiveTO,u8_SetDriverSeatBeltCmdTO,u8_SetRFPressIndiTO,u8_SetLFPressIndiTO,u8_SetRRPressIndiTO,u8_SetLRPressIndiTO,u8_SetsigAmbAirTTO,u8_SetAPS_PwrReqAvail_staTO,u8_SetDKC_PDkeyAreaRAPS_StaTO,u8_SetDKC_ParkingMode_CmdTO,u8_SetP_UID_LowPowerTO,u8_SetDr_SeatStaTO,u8_SetVCU_RAPSErrLv2_flgTO,u8_SetVCU_RAPSErrLv3_flgTO,u8_SetIVI_UserTakeOver_APS_StaTO)  InputArgumentSpecifications=uint8(1), uint8(1), uint8(1), uint8(1), uint8(1), uint8(1), uint8(1), uint8(1), uint8(1), uint8(1), uint8(1), uint8(1), uint8(1), uint8(1), uint8(1), uint8(1), uint8(1), uint8(1), uint8(1), uint8(1), uint8(1), uint8(1), uint8(1), uint8(1), uint8(1), uint8(1), uint8(1), uint8(1), uint8(1), uint8(1), uint8(1), uint8(1), uint8(1), uint8(1), uint8(1), uint8(1), uint8(1), uint8(1), uint8(1), uint8(1), uint8(1), uint8(1), uint8(1), uint8(1), uint8(1), uint8(1), uint8(1), uint8(1), uint8(1), uint8(1), uint8(1), uint8(1), uint8(1), uint8(1), uint8(1), uint8(1), uint8(1), uint8(1), uint8(1), uint8(1), uint8(1), uint8(1), uint8(1), uint8(1), uint8(1), uint8(1), uint8(1), uint8(1), uint8(1)
  R_NVMReadCDD_Inner_NVM_ReadOperation : Subsystem
  R_NVMWriteCDD_Inner_NVM_WriteOperation : Subsystem
  R_UDSCDD_CSOP_DdmClearDTCNotification : FunctionCaller  FunctionPrototype=u8_ClearDTCcmd = R_UDSCDD_CSOP_DdmClearDTCNotification()  OutputArgumentSpecifications=uint8(1)
  R_UDSCDD_CSOP_DdmRestartOperationCycle : Subsystem
  R_UDSCDD_CSOP_SetDTCStatus : Subsystem
  R_WDGCDD_CSOP_Call_WDG_AppEnd : Subsystem
  R_WDGCDD_CSOP_Call_WDG_AppStart : Subsystem
  R_WDGCDD_CSOP_Call_Watchdog : Subsystem
  Real_DetectChange : hcu_lib/Basic_Blocks/Real_DetectChange
  Subsystem : Subsystem
  Subsystem1 : Subsystem
  Subsystem3 : Subsystem
  Subsystem4 : Subsystem
  Subsystem5 : Subsystem
  Subsystem6 : Subsystem
  Subsystem7 : Subsystem
  Terminator{,1..7} (8 alike) : Terminator
  Terminator_11 : Terminator
  Unit Delay{,1..3} (4 alike) : UnitDelay  SampleTime=-1  HasFrameUpgradeWarning=on
  detect_Increase : simulink/Logic and Bit Operations/Detect Increase  vinit=0.0  OutDataTypeStr=boolean
  detect_change : simulink/Logic and Bit Operations/Detect Change  vinit=0  OutDataTypeStr=boolean
  detect_change1 : simulink/Logic and Bit Operations/Detect Change  vinit=0  OutDataTypeStr=boolean
  hcu_main_sched : Stateflow chart  TreatAsAtomicUnit=on
      settings: PortSchema="{\"entries\":[{\"content\":{\"sides\":[{\"content\":{\"connectorIds\":[\"In1\",\"In2\"]},\"type\":\"ConnectorPlacement.EquallySpacedRectSide\",\"uuid\":\"b7e373d4-7b92-4563-a962-1396bf0d3836\"},{\"content\":{\"connectorIds\":[\"Out1\",\"Out16\",\"Out2\",\"Out3\",\"Out4\",\"Out5\",\"Out6\",\"Out7\",\"Out8\",\"Out9\",\"Out10\",\"Out11\",\"Out12\",\"Out13\",\"Out17\",\"Out14\",\"Out15\"],\"side\":\"RIGHT\"},\"type\":\"ConnectorPlacement.EquallySpacedRectSide\",\"uuid\":\"9162eed8-852f-437e-b7a7-3f514daa5dad\"},{\"content\":{\"connectorIds\":[],\"side\":\"TOP\"},\"type\":\"ConnectorPlacement.EquallySpacedRectSide\",\"uuid\":\"4ba5874d-9ced-4b78-a5b9-28a1ade43d03\"}]},\"type\":\"ConnectorPlacement.EquallySpacedConnector\",\"uuid\":\"986bc96e-cdd1-4540-b0f0-d43c4f1d98ba\"}],\"packageUris\":[\"http://schema.mathworks.com/mf0/Connector/R2020b\"],\"version\":\"1.0\"}"
  P_CAN1_FD1_BCM1_CAN1_SG_FD1_BCM1_write : Outport
  P_CAN1_FD1_VCU1_CAN1_SG_FD1_VCU1_write : Outport  Port=2
  P_CAN1_FD1_VMC1_CAN1_SG_FD1_VMC1_write : Outport  Port=3
  P_CAN2_FD2_CE100_0_CAN2_SG_FD2_CE100_0_write : Outport  Port=4
  P_CAN2_FD2_CE200_1_CAN2_SG_FD2_CE200_1_write : Outport  Port=5
  P_CAN2_GW2_CE100_0_CAN2_SG_GW2_CE100_0_write : Outport  Port=6
  P_CAN2_GW2_CE200_0_CAN2_SG_GW2_CE200_0_write : Outport  Port=7
  P_CAN3_FD3_BCM1_CAN3_SG_FD3_BCM1_write : Outport  Port=8
  P_CAN3_FD3_THCM2_CAN3_SG_FD3_THCM2_write : Outport  Port=9
  P_CAN3_FD3_V2L1_CAN3_SG_FD3_V2L1_write : Outport  Port=10
  P_CAN4_FD4_CE100_1_CAN4_SG_FD4_CE100_1_write : Outport  Port=11
  P_CAN4_FD4_CE200_0_CAN4_SG_FD4_CE200_0_write : Outport  Port=12
  P_CAN4_GW4_CE100_0_CAN4_SG_GW4_CE100_0_write : Outport  Port=13
  P_CAN5_FD5_CE100_0_CAN5_SG_FD5_CE100_0_write : Outport  Port=14
  P_CAN5_FD5_Debug1_CAN5_SG_FD5_Debug1_write : Outport  Port=15
  P_CAN5_FD5_Debug2_CAN5_SG_FD5_Debug2_write : Outport  Port=16
  P_CAN6_FD6_BCM1_CAN6_SG_FD6_BCM1_write : Outport  Port=17
  P_CAN6_FD6_VCU1_CAN6_SG_FD6_VCU1_write : Outport  Port=18
  P_CAN6_FD6_VMC1_CAN6_SG_FD6_VMC1_write : Outport  Port=19
  P_CAN6_GW6_CE100_0_CAN6_SG_GW6_CE100_0_write : Outport  Port=20
  IRV_ms10_CAN1_SG_FD1_APS3_write : Outport  Port=21  OutDataTypeStr=Bus: DT_CAN1_SG_FD1_APS3  PortDimensions=1  BusOutputAsStruct=on
  IRV_ms10_CAN1_SG_FD1_VCU2_write : Outport  Port=22  OutDataTypeStr=Bus: DT_CAN1_SG_FD1_VCU2  PortDimensions=1  BusOutputAsStruct=on
  IRV_ms10_CAN1_SG_FD1_VCU3_write : Outport  Port=23  OutDataTypeStr=Bus: DT_CAN1_SG_FD1_VCU3  PortDimensions=1  BusOutputAsStruct=on
  IRV_ms10_CAN1_SG_VMC_FCM1_write : Outport  Port=24  OutDataTypeStr=Bus: DT_CAN1_SG_VMC_FCM1  PortDimensions=1  BusOutputAsStruct=on
  IRV_ms10_CAN3_SG_FD3_VCU0_write : Outport  Port=25  OutDataTypeStr=Bus: DT_CAN3_SG_FD3_VCU0  PortDimensions=1  BusOutputAsStruct=on
  IRV_ms10_CAN3_SG_FD3_VCU2_write : Outport  Port=26  OutDataTypeStr=Bus: DT_CAN3_SG_FD3_VCU2  PortDimensions=1  BusOutputAsStruct=on
  IRV_ms10_CAN3_SG_FD3_VCU2_toNIDEC_write : Outport  Port=27  OutDataTypeStr=Bus: DT_CAN3_SG_FD3_VCU2_toNIDEC  PortDimensions=1  BusOutputAsStruct=on
  IRV_ms10_CAN3_SG_FD3_VCU5_write : Outport  Port=28  OutDataTypeStr=Bus: DT_CAN3_SG_FD3_VCU5  PortDimensions=1  BusOutputAsStruct=on
  IRV_ms10_CAN3_SG_GW_ESC1_toNIDEC_write : Outport  Port=29  OutDataTypeStr=Bus: DT_CAN3_SG_GW_ESC1_toNIDEC  PortDimensions=1  BusOutputAsStruct=on
  IRV_ms10_CAN5_SG_FD5_Debug3_write : Outport  Port=30  OutDataTypeStr=Bus: DT_CAN5_SG_FD5_Debug3  PortDimensions=1  BusOutputAsStruct=on
  IRV_ms10_CAN6_SG_FD6_APS3_write : Outport  Port=31  OutDataTypeStr=Bus: DT_CAN6_SG_FD6_APS3  PortDimensions=1  BusOutputAsStruct=on
  IRV_ms10_CAN6_SG_FD6_VCU2_write : Outport  Port=32  OutDataTypeStr=Bus: DT_CAN6_SG_FD6_VCU2  PortDimensions=1  BusOutputAsStruct=on
  IRV_ms100_CAN1_SG_FD1_THCM1_write : Outport  Port=33  OutDataTypeStr=Bus: DT_CAN1_SG_FD1_THCM1  PortDimensions=1  BusOutputAsStruct=on
  IRV_ms100_CAN3_SG_FD3_THCM1_write : Outport  Port=34  OutDataTypeStr=Bus: DT_CAN3_SG_FD3_THCM1  PortDimensions=1  BusOutputAsStruct=on
  IRV_ms1000_CAN3_SG_GW_IVI6_toNIDEC_write : Outport  Port=35  OutDataTypeStr=Bus: DT_CAN3_SG_GW_IVI6_toNIDEC  PortDimensions=1  BusOutputAsStruct=on
  IRV_ms20_CAN1_SG_FD1_APS2_write : Outport  Port=36  OutDataTypeStr=Bus: DT_CAN1_SG_FD1_APS2  PortDimensions=1  BusOutputAsStruct=on
  IRV_ms20_CAN2_SG_FD2_C20_0_write : Outport  Port=37  OutDataTypeStr=Bus: DT_CAN2_SG_FD2_C20_0  PortDimensions=1  BusOutputAsStruct=on
  IRV_ms500_CAN1_SG_FD1_VMC2_write : Outport  Port=38  OutDataTypeStr=Bus: DT_CAN1_SG_FD1_VMC2  PortDimensions=1  BusOutputAsStruct=on
  IRV_ms5000_CAN2_SG_FD2_Version_write : Outport  Port=39  OutDataTypeStr=Bus: DT_CAN2_SG_FD2_Version  PortDimensions=1  BusOutputAsStruct=on
  IRV_E2E_CAN3_SG_FD3_VCU1_write : Outport  Port=40  OutDataTypeStr=Bus: DT_CAN3_SG_FD3_VCU1  PortDimensions=1  BusOutputAsStruct=on
  IRV_E2E_CAN3_SG_FD3_VCU1_toNIDEC_write : Outport  Port=41  OutDataTypeStr=Bus: DT_CAN3_SG_FD3_VCU1_toNIDEC  PortDimensions=1  BusOutputAsStruct=on
  IRV_E2E_CAN4_SG_FD4_CE100_0_write : Outport  Port=42  OutDataTypeStr=Bus: DT_CAN4_SG_FD4_CE100_0  PortDimensions=1  BusOutputAsStruct=on
  IRV_f32_ApsOutVehSpdSig_write : Outport  Port=43  OutDataTypeStr=single  PortDimensions=1
  IRV_u8Array256_NvmWriteArray_write : Outport  Port=44  OutDataTypeStr=uint8  PortDimensions=256
  IRV_u8_ApsOutGearPosnSig_write : Outport  Port=45  OutDataTypeStr=uint8  PortDimensions=1
  IRV_u8_ApsOutSendChrgPlugSta_write : Outport  Port=46  OutDataTypeStr=uint8  PortDimensions=1
  IRV_u8_ApsOutSetFrSensorOnCmd_write : Outport  Port=47  OutDataTypeStr=uint8  PortDimensions=1
  IRV_u8_ApsOutSetFrSensorSwTOCmd_write : Outport  Port=48  OutDataTypeStr=uint8  PortDimensions=1
  IRV_u8_ApsOutSetVehSpdTOCmd_write : Outport  Port=49  OutDataTypeStr=uint8  PortDimensions=1
  wires:
  IRV_u16Array4_ApsInDist_read/1 -> [u16Array4_ApsInDist]
  IRV_u8Array12_ApsInUssSta_read/1 -> [u8Array12_ApsInUssSta]
  IRV_u8Array256_NvmReadArray_read/1 -> [u8Array256_NvmReadArray]
  IRV_u8Array8_ApsInLevel_read/1 -> [u8Array8_ApsInLevel]
  IRV_u8Array8_PasInDist_read/1 -> [u8Array8_PasInDist]
  IRV_u8Array9_TPMSData_read/1 -> [u8Array9_TPMSData]
  IRV_u8_ApsInPASChime_read/1 -> [u8_ApsInPASChime]
  IRV_u8_ApsInSensorLayout_read/1 -> [u8_ApsInSensorLayout]
  IRV_u8_ApsInSysFailSta_read/1 -> [u8_ApsInSysFailSta]
  IRV_u8_ApsInSysMode_read/1 -> [u8_ApsInSysMode]
  IRV_u8_CTDSW_read/1 -> [u8_CTDSW]
  IRV_u8_CrashSignal_read/1 -> [u8_CrashSignal]
  IRV_u8_DrDoorSW_read/1 -> [u8_DrDoorSW]
  IRV_u8_HazardSW_read/1 -> [u8_HazardSW]
  IRV_u8_HoodSW_read/1 -> [u8_HoodSW]
  IRV_u8_PsDoorSW_read/1 -> [u8_PsDoorSW]
  IRV_u8_RLDoorSW_read/1 -> [u8_RLDoorSW]
  IRV_u8_RRDoorSW_read/1 -> [u8_RRDoorSW]
  IRV_u8_SeatSW_read/1 -> [u8_SeatSW]
  IRV_u8_TPMSDataInSta_read/1 -> [u8_TPMSDataInSta]
  IRV_u8_TailgateSW_read/1 -> [u8_TailgateSW]
  IRV_u8_TrunkHanSW_read/1 -> [u8_TrunkHanSW]
  [f32_ApsOutVehSpdSig] -> IRV_f32_ApsOutVehSpdSig_write/1
  [u8Array256_NvmWriteArray] -> IRV_u8Array256_NvmWriteArray_write/1
  [u8_ApsOutGearPosnSig] -> IRV_u8_ApsOutGearPosnSig_write/1
  [u8_ApsOutSendChrgPlugSta] -> IRV_u8_ApsOutSendChrgPlugSta_write/1
  [u8_ApsOutSetFrSensorOnCmd] -> IRV_u8_ApsOutSetFrSensorOnCmd_write/1
  [u8_ApsOutSetFrSensorSwTOCmd] -> IRV_u8_ApsOutSetFrSensorSwTOCmd_write/1
  [u8_ApsOutSetVehSpdTOCmd] -> IRV_u8_ApsOutSetVehSpdTOCmd_write/1
  R_HALINCDD_CSOP_AnyNmID/1 -> [u8_AnyNMID]
  R_HALINCDD_CSOP_CAN1BusOff/1 -> [u8_CAN1BusOff]
  R_HALINCDD_CSOP_CAN2BusOff/1 -> [u8_CAN2BusOff]
  R_HALINCDD_CSOP_CAN3BusOff/1 -> [u8_CAN3BusOff]
  R_HALINCDD_CSOP_CAN4BusOff/1 -> [u8_CAN4BusOff]
  R_HALINCDD_CSOP_CAN5BusOff/1 -> [u8_CAN5BusOff]
  Constant/1 -> R_HALINCDD_CSOP_DIDgetDKCdata/1
  Constant1/1 -> R_HALINCDD_CSOP_DIDgetDKCdata/2
  R_HALINCDD_CSOP_DIDgetDKCdata/1 -> [u8_DidStaDKC]
  R_HALINCDD_CSOP_DIDgetDKCdata/2 -> [u8Array8_DidDataDKC]
  Constant2/1 -> R_HALINCDD_CSOP_DIDgetXWDdata/1
  Constant3/1 -> R_HALINCDD_CSOP_DIDgetXWDdata/2
  R_HALINCDD_CSOP_DIDgetXWDdata/1 -> [u8_DidStaXWD]
  R_HALINCDD_CSOP_DIDgetXWDdata/2 -> [u8_DidDataXWD]
  R_HALINCDD_CSOP_GetAcoreReadyToSleep/1 -> [s8_AcoreReadyToSleep]
  R_HALINCDD_CSOP_GetAcoreRebootCmd/1 -> [u8_AcoreRebootCmd]
  R_HALINCDD_CSOP_GetAuxBattVoltage/1 -> [u16_AuxBattVol100mV]
  R_HALINCDD_CSOP_GetBootReason/1 -> [u8_BootReason]
  R_HALINCDD_CSOP_GetEvccAplusPwrUpReq/1 -> [u8_EvccAplusPwrUpReq]
  R_HALINCDD_CSOP_GetNmState/1 -> [u8_CurrentNMState]
  R_HALINCDD_CSOP_GetNvmProtectState/1 -> [u8_NvmProtectSta]
  R_HALINCDD_CSOP_GetSWID/1 -> [u8Array33_SWID]
  R_HALINCDD_CSOP_GetVinpAllowMoveThdOta/1 -> [u8_AllowMovThdOTA]
  R_HALINCDD_CSOP_GetVinpPwrReqOta/1 -> [u8_PwrReqOTA]
  R_HALINCDD_CSOP_GetWISR/1 -> [u32_WISR]
  R_HALINCDD_CSOP_HALINCDD_DIRECT/1 -> [u8_BrakeSW]
  R_HALINCDD_CSOP_HALINCDD_DIRECT/2 -> [u8_BrakeLamp]
  R_HALINCDD_CSOP_HALINCDD_DIRECT/3 -> [u16_Pedal1Vol]
  R_HALINCDD_CSOP_HALINCDD_DIRECT/4 -> [u16_Pedal2Vol]
  R_HALINCDD_CSOP_HALINCDD_DIRECT/5 -> [u16_Pedal1Ref5V]
  R_HALINCDD_CSOP_HALINCDD_DIRECT/6 -> [u16_Pedal2Ref5V]
  R_HALINCDD_u8Array4_HWID/1 -> [u8Array4_HWID]
  R_HALIN_APS_CSOP_ApsGetData/1 -> [u8_GetAPS_Progress_PCT]
  R_HALIN_APS_CSOP_ApsGetData/2 -> [u8_GetAPS_RQ_Display]
  R_HALIN_APS_CSOP_ApsGetData/3 -> [u8_GetAPS_SW_Ver]
  R_HALIN_APS_CSOP_ApsGetData/4 -> [u8_GetAPS_HW_Ver]
  R_HALIN_APS_CSOP_ApsGetData/5 -> [u8_GetAPS_ExitCondition]
  R_HALIN_APS_CSOP_ApsGetData/6 -> [f32_GetAPS_Angle_Target]
  R_HALIN_APS_CSOP_ApsGetData/7 -> [u8_GetAPS_Sta_System]
  R_HALIN_APS_CSOP_ApsGetData/8 -> [u8_GetAPS_V_Rq_EPAS_Ctrl]
  R_HALIN_APS_CSOP_ApsGetData/9 -> [u8_GetAPS_Rq_EPAS_Ctrl]
  R_HALIN_APS_CSOP_ApsGetData/10 -> [u8_GetAPS_Req]
  R_HALIN_APS_CSOP_ApsGetData/11 -> [f32_GetAPS_DecReq]
  R_HALIN_APS_CSOP_ApsGetData/12 -> [u8_GetAPS_DecReq_A]
  R_HALIN_APS_CSOP_ApsGetData/13 -> [f32_GetAPS_SpeedCmd]
  R_HALIN_APS_CSOP_ApsGetData/14 -> [u8_GetAPS_ShftPosnReq]
  R_HALIN_APS_CSOP_ApsGetData/15 -> [u8_GetAPS_VMC_Req_A]
  R_HALIN_APS_CSOP_ApsGetData/16 -> [u8_GetCAAS_Sta]
  R_HALIN_APS_CSOP_ApsGetData/17 -> [u8_GetCAAS_VMC_Req_A]
  R_HALIN_APS_CSOP_ApsGetData/18 -> [u8_GetAPS_PwrReq_cmd]
  R_HALIN_APS_CSOP_ApsGetData/19 -> [u8_GetRAPS_BCM_LockReq_Cmd]
  R_HALIN_APS_CSOP_ApsGetData/20 -> [u8_GetRAPS_BCM_Lamp_Cmd]
  R_HALIN_APS_CSOP_ApsGetData/21 -> [u8_GetRAPS_ErrWarn_Sta]
  R_HALIN_APS_CSOP_ApsGetData/22 -> [u8_GetRAPS_ErrLv1_flg]
  R_HALIN_IMU_CSOP_IMUGetSixAxisVal/1 -> [s16_IMUSixAxisVal]
  R_HALIN_IMU_CSOP_IMUGetSixAxisVal/2 -> [u8_IMUSixAxisValSta]
  R_UDSCDD_CSOP_DdmClearDTCNotification/1 -> [u8_ClearDTCcmd]
  Bus Selector17/1 -> detect_change1/1, Data Type Conversion/1  "<VOUTP_IVIRST_flg>"
  Data Type Conversion1/1 -> R_HALOUTCDD_CSOP_SetSysPwrStat/1
  Bus Selector11/1 -> Data Type Conversion1/1  "<VOUTP_SysPowerMode_enum>"
  Data Type Conversion2/1 -> R_HALOUTCDD_CSOP_AppNmStateReq/1(WakeReq)
  Data Type Conversion3/1 -> R_HALOUTCDD_CSOP_AppNmStateReq/2(SleepReq)
  NOT/1 -> Data Type Conversion3/1
  detect_change/1 -> R_HALOUTCDD_CSOP_AppNmStateReq/Enable
  Bus Selector10/1 -> Data Type Conversion2/1, NOT/1, detect_change/1  "<VOUTP_NetworkReq_flg>"
  Bus Selector12/1 -> R_NVMWriteCDD_Inner_NVM_WriteOperation/Enable  "<VOUTP_NvWriteReqRisingEdge_flg>"
  Data Type Conversion4/1 -> R_HALOUTCDD_CSOP_SleepRequest/2(WakeUpTime)
  Bus Selector16/1 -> Data Type Conversion4/1  "<VOUTP_FdcSlpTime_sec>"
  Bus Selector13/1 -> R_HALOUTCDD_CSOP_SleepRequest/Enable  "<VOUTP_FdcSlpReqRisingEdge_flg>"
  Unit Delay/1 -> R_WDGCDD_CSOP_Call_WDG_AppEnd/Enable
  Bus Selector14/1 -> Unit Delay/1  "<VOUTP_FdcSlpReqRisingEdge_flg>"
  Unit Delay1/1 -> R_FDCCDD_Inner_CSOP_FDC_AppCallSleep/Enable
  Unit Delay2/1 -> Unit Delay1/1
  Bus Selector15/1 -> Unit Delay2/1  "<VOUTP_FdcSlpReqRisingEdge_flg>"
  [Header_Array] -> R_UDSCDD_CSOP_SetDTCStatus/1(Header_Array)
  [DTC_Array] -> R_UDSCDD_CSOP_SetDTCStatus/2(DTC_Array)
  [DTC_Trigger] -> R_UDSCDD_CSOP_SetDTCStatus/Enable
  [trig_Read_NVM_00] -> R_NVMReadCDD_Inner_NVM_ReadOperation/Trigger
  [trig_WDG] -> R_WDGCDD_CSOP_Call_Watchdog/Trigger
  detect_Increase/1 -> R_WDGCDD_CSOP_Call_WDG_AppStart/Enable
  Constant4/1 -> detect_Increase/1
  [trig_ReadIMUOffset_00] -> R_HALIN_IMU_CSOP_IMUGetOffsetVal/Trigger
  R_HALIN_IMU_CSOP_IMUGetOffsetVal/1(Out1) -> [s16_IMUOffsetVal]
  R_HALIN_IMU_CSOP_IMUGetOffsetVal/2(Out2) -> [u8_IMUOffsetValSta]
  [E2E_CAN3_VCU1_Trigger] -> HALOUT_AFTER/1(E2E_CAN3_VCU1_Trigger)
  [E2E_CAN3_VCU1_toNIDEC_Trigger] -> HALOUT_AFTER/2(E2E_CAN3_VCU1_Trigger_toNIDEC)
  [E2E_CAN4_VCU1_Trigger] -> HALOUT_AFTER/3(E2E_CAN4_VCU1_Trigger)
  [trig_HAL_OUTAFTER_50_1] -> HALOUT_AFTER/Trigger
  Data Type Conversion85/1 -> R_HALOUT_APS_CSOP_ApsSetTimeout/49
  Ground_19/1 -> Data Type Conversion113/1
  Data Type Conversion52/1 -> R_HALOUT_APS_CSOP_ApsSetTimeout/20
  Data Type Conversion88/1 -> R_HALOUT_APS_CSOP_ApsSetTimeout/53
  Bus Selector4/42 -> Data Type Conversion76/1  "<VOUTP_ESCAPSStaTimeOut_flg>"
  Bus Selector4/15 -> Data Type Conversion47/1  "<VOUTP_RFPulseCountVTimeOut_flg>"
  Bus Selector4/25 -> Data Type Conversion58/1  "<VOUTP_SASAngleTimeOut_flg>"
  Bus Selector4/13 -> Data Type Conversion55/1  "<VOUTP_RRWhlRotDirTimeOut_flg>"
  Bus Selector4/52 -> Data Type Conversion87/1  "<VOUTP_CAASSwTimeOut_flg>"
  Ground1/1 -> Data Type Conversion91/1
  Bus Selector4/9 -> Data Type Conversion41/1  "<VOUTP_RRRawWhlSpeedVTimeOut_flg>"
  Bus Selector4/44 -> Data Type Conversion77/1  "<VOUTP_EPBExtApplyAvailTimeOut_flg>"
  Bus Selector4/4 -> Data Type Conversion19/1  "<VOUTP_LRRawWhlSpeedTimeOut_flg>"
  Bus Selector4/55 -> Data Type Conversion84/1  "<VOUTP_TCSActiveTimeOut_flg>"
  Bus Selector4/33 -> Data Type Conversion75/1  "<VOUTP_LongAccelTimeOut_flg>"
  Bus Selector4/54 -> Data Type Conversion81/1  "<VOUTP_ABSActiveTimeOut_flg>"
  Bus Selector4/58 -> Terminator2/1  "<VOUTP_LFPressIndi_enum>"
  Bus Selector4/60 -> Terminator4/1  "<VOUTP_LRPressIndi_enum>"
  Ground_23/1 -> Data Type Conversion116/1
  Bus Selector4/27 -> Data Type Conversion60/1  "<VOUTP_SASSpeedValidTimeOut_flg>"
  Ground_26/1 -> Data Type Conversion114/1
  Bus Selector4/3 -> Data Type Conversion50/1  "<VOUTP_RFRawWhlSpeedTimeOut_flg>"
  Bus Selector4/36 -> Data Type Conversion68/1  "<VOUTP_LatAccelVTimeOut_flg>"
  Bus Selector4/16 -> Data Type Conversion48/1  "<VOUTP_LRPulseCountVTimeOut_flg>"
  Bus Selector4/29 -> Data Type Conversion61/1  "<VOUTP_SASVTimeOut_flg>"
  Bus Selector4/14 -> Data Type Conversion46/1  "<VOUTP_LFPulseCountVTimeOut_flg>"
  Bus Selector4/19 -> Data Type Conversion51/1  "<VOUTP_RFPulseCountTimeOut_flg>"
  Bus Selector4/6 -> Data Type Conversion39/1  "<VOUTP_LFRawWhlSpeedVTimeOut_flg>"
  Bus Selector4/40 -> Data Type Conversion72/1  "<VOUTP_BrkSwVTimeOut_flg>"
  Ground4/1 -> Data Type Conversion94/1
  Bus Selector4/10 -> Data Type Conversion42/1  "<VOUTP_LFWhlRotDirTimeOut_flg>"
  Ground2/1 -> Data Type Conversion92/1
  Data Type Conversion81/1 -> R_HALOUT_APS_CSOP_ApsSetTimeout/54
  Data Type Conversion114/1 -> R_HALOUT_APS_CSOP_ApsSetTimeout/69
  Data Type Conversion115/1 -> R_HALOUT_APS_CSOP_ApsSetTimeout/68
  Data Type Conversion80/1 -> R_HALOUT_APS_CSOP_ApsSetTimeout/1
  Data Type Conversion43/1 -> R_HALOUT_APS_CSOP_ApsSetTimeout/11
  Data Type Conversion40/1 -> R_HALOUT_APS_CSOP_ApsSetTimeout/7
  Data Type Conversion39/1 -> R_HALOUT_APS_CSOP_ApsSetTimeout/6
  Data Type Conversion110/1 -> R_HALOUT_APS_CSOP_ApsSetTimeout/66
  Data Type Conversion38/1 -> R_HALOUT_APS_CSOP_ApsSetTimeout/5
  Data Type Conversion61/1 -> R_HALOUT_APS_CSOP_ApsSetTimeout/29
  Data Type Conversion112/1 -> R_HALOUT_APS_CSOP_ApsSetTimeout/64
  Data Type Conversion90/1 -> R_HALOUT_APS_CSOP_ApsSetTimeout/43
  Data Type Conversion42/1 -> R_HALOUT_APS_CSOP_ApsSetTimeout/10
  Bus Selector4/23 -> Data Type Conversion70/1  "<VOUTP_DriIntendTimeOut_flg>"
  Data Type Conversion86/1 -> R_HALOUT_APS_CSOP_ApsSetTimeout/51
  Ground_24/1 -> Data Type Conversion115/1
  Data Type Conversion63/1 -> R_HALOUT_APS_CSOP_ApsSetTimeout/31
  Data Type Conversion53/1 -> R_HALOUT_APS_CSOP_ApsSetTimeout/21
  Data Type Conversion56/1 -> R_HALOUT_APS_CSOP_ApsSetTimeout/22
  Data Type Conversion59/1 -> R_HALOUT_APS_CSOP_ApsSetTimeout/26
  Data Type Conversion83/1 -> R_HALOUT_APS_CSOP_ApsSetTimeout/48
  Data Type Conversion76/1 -> R_HALOUT_APS_CSOP_ApsSetTimeout/42
  Data Type Conversion55/1 -> R_HALOUT_APS_CSOP_ApsSetTimeout/13
  Data Type Conversion94/1 -> R_HALOUT_APS_CSOP_ApsSetTimeout/58
  Data Type Conversion69/1 -> R_HALOUT_APS_CSOP_ApsSetTimeout/37
  Data Type Conversion78/1 -> R_HALOUT_APS_CSOP_ApsSetTimeout/45
  Data Type Conversion50/1 -> R_HALOUT_APS_CSOP_ApsSetTimeout/3
  Bus Selector4/12 -> Data Type Conversion45/1  "<VOUTP_LRWhlRotDirTimeOut_flg>"
  Data Type Conversion72/1 -> R_HALOUT_APS_CSOP_ApsSetTimeout/40
  Data Type Conversion116/1 -> R_HALOUT_APS_CSOP_ApsSetTimeout/67
  Bus Selector4/1 -> Data Type Conversion80/1  "<VOUTP_BrkPedalPosTimeOut_flg>"
  Data Type Conversion71/1 -> R_HALOUT_APS_CSOP_ApsSetTimeout/39
  Data Type Conversion60/1 -> R_HALOUT_APS_CSOP_ApsSetTimeout/27
  Data Type Conversion70/1 -> R_HALOUT_APS_CSOP_ApsSetTimeout/23
  Bus Selector4/41 -> Data Type Conversion73/1  "<VOUTP_ESCStandstillTimeOut_flg>"
  Data Type Conversion54/1 -> R_HALOUT_APS_CSOP_ApsSetTimeout/18
  Bus Selector4/34 -> Data Type Conversion66/1  "<VOUTP_MCPressureTimeOut_flg>"
  Data Type Conversion62/1 -> R_HALOUT_APS_CSOP_ApsSetTimeout/30
  Data Type Conversion67/1 -> R_HALOUT_APS_CSOP_ApsSetTimeout/35
  Data Type Conversion44/1 -> R_HALOUT_APS_CSOP_ApsSetTimeout/8
  Data Type Conversion64/1 -> R_HALOUT_APS_CSOP_ApsSetTimeout/28
  Data Type Conversion65/1 -> R_HALOUT_APS_CSOP_ApsSetTimeout/32
  Data Type Conversion45/1 -> R_HALOUT_APS_CSOP_ApsSetTimeout/12
  Data Type Conversion49/1 -> R_HALOUT_APS_CSOP_ApsSetTimeout/17
  Data Type Conversion79/1 -> R_HALOUT_APS_CSOP_ApsSetTimeout/46
  Data Type Conversion66/1 -> R_HALOUT_APS_CSOP_ApsSetTimeout/34
  Bus Selector4/47 -> Data Type Conversion82/1  "<VOUTP_AVMparkingcancelTimeOut_flg>"
  Data Type Conversion123/1 -> R_HALOUT_APS_CSOP_ApsSetTimeout/2
  Bus Selector4/45 -> Data Type Conversion78/1  "<VOUTP_EPBErrStaTimeOut_flg>"
  Ground_21/1 -> Data Type Conversion111/1
  Bus Selector4/57 -> Terminator1/1  "<VOUTP_RFPressIndi_enum>"
  Bus Selector4/48 -> Data Type Conversion83/1  "<VOUTP_AVMparkingexcuteTimeOut_flg>"
  Data Type Conversion46/1 -> R_HALOUT_APS_CSOP_ApsSetTimeout/14
  Bus Selector4/31 -> Data Type Conversion63/1  "<VOUTP_YawRateTimeOut_flg>"
  Data Type Conversion47/1 -> R_HALOUT_APS_CSOP_ApsSetTimeout/15
  Bus Selector4/22 -> Data Type Conversion56/1  "<VOUTP_ShifterHandleCmdTimeOut_flg>"
  Bus Selector4/2 -> Data Type Conversion123/1  "<VOUTP_LFRawWhlSpeedTimeOut_flg>"
  Bus Selector4/56 -> Data Type Conversion89/1  "<VOUTP_DriverSeatBeltCmdTimeOut_flg>"
  Ground5/1 -> Data Type Conversion106/1
  Bus Selector4/17 -> Data Type Conversion49/1  "<VOUTP_RRPulseCountVTimeOut_flg>"
  Bus Selector4/20 -> Data Type Conversion52/1  "<VOUTP_LRPulseCountTimeOut_flg>"
  Bus Selector4/32 -> Data Type Conversion65/1  "<VOUTP_LatAccelTimeOut_flg>"
  Data Type Conversion68/1 -> R_HALOUT_APS_CSOP_ApsSetTimeout/36
  Data Type Conversion111/1 -> R_HALOUT_APS_CSOP_ApsSetTimeout/65
  Bus Selector4/53 -> Data Type Conversion88/1  "<VOUTP_IVIScreenTimeOut_flg>"
  Data Type Conversion57/1 -> R_HALOUT_APS_CSOP_ApsSetTimeout/24
  Ground_22/1 -> Data Type Conversion110/1
  Data Type Conversion113/1 -> R_HALOUT_APS_CSOP_ApsSetTimeout/63
  Bus Selector4/11 -> Data Type Conversion43/1  "<VOUTP_RFWhlRotDirTimeOut_flg>"
  Bus Selector4/28 -> Data Type Conversion64/1  "<VOUTP_SASCALTimeOut_flg>"
  Data Type Conversion93/1 -> R_HALOUT_APS_CSOP_ApsSetTimeout/59
  Bus Selector4/43 -> Data Type Conversion90/1  "<VOUTP_EPBExtReleaseAvailTimeOut_flg>"
  Bus Selector4/38 -> Data Type Conversion74/1  "<VOUTP_MCPressureVTimeOut_flg>"
  Data Type Conversion73/1 -> R_HALOUT_APS_CSOP_ApsSetTimeout/41
  Ground_18/1 -> Data Type Conversion109/1
  Bus Selector4/35 -> Data Type Conversion67/1  "<VOUTP_YawRateVTimeOut_flg>"
  Data Type Conversion87/1 -> R_HALOUT_APS_CSOP_ApsSetTimeout/52
  Data Type Conversion89/1 -> R_HALOUT_APS_CSOP_ApsSetTimeout/56
  Data Type Conversion95/1 -> R_HALOUT_APS_CSOP_ApsSetTimeout/50
  Data Type Conversion41/1 -> R_HALOUT_APS_CSOP_ApsSetTimeout/9
  Data Type Conversion77/1 -> R_HALOUT_APS_CSOP_ApsSetTimeout/44
  Data Type Conversion48/1 -> R_HALOUT_APS_CSOP_ApsSetTimeout/16
  Data Type Conversion109/1 -> R_HALOUT_APS_CSOP_ApsSetTimeout/62
  Data Type Conversion91/1 -> R_HALOUT_APS_CSOP_ApsSetTimeout/61
  [BOUTP_outputs] -> Bus Selector4/1
  Data Type Conversion19/1 -> R_HALOUT_APS_CSOP_ApsSetTimeout/4
  Data Type Conversion84/1 -> R_HALOUT_APS_CSOP_ApsSetTimeout/55
  Bus Selector4/7 -> Data Type Conversion40/1  "<VOUTP_RFRawWhlSpeedVTimeOut_flg>"
  Bus Selector4/59 -> Terminator3/1  "<VOUTP_RRPressIndi_enum>"
  Bus Selector4/61 -> Terminator5/1  "<VOUTP_sigAmbAirT_C>"
  Bus Selector4/5 -> Data Type Conversion38/1  "<VOUTP_RRRawWhlSpeedTimeOut_flg>"
  Bus Selector4/26 -> Data Type Conversion59/1  "<VOUTP_SASSpeedTimeOut_flg>"
  Bus Selector4/30 -> Data Type Conversion62/1  "<VOUTP_GRADETimeOut_flg>"
  Bus Selector4/51 -> Data Type Conversion86/1  "<VOUTP_IVIStatusTimeOut_flg>"
  Bus Selector4/46 -> Data Type Conversion79/1  "<VOUTP_EPBStaTimeOut_flg>"
  Ground3/1 -> Data Type Conversion93/1
  Data Type Conversion51/1 -> R_HALOUT_APS_CSOP_ApsSetTimeout/19
  Bus Selector4/50 -> Data Type Conversion95/1  "<VOUTP_AVMErrSTATimeOut_flg>"
  Bus Selector4/49 -> Data Type Conversion85/1  "<VOUTP_AVMParkingmodeTimeOut_flg>"
  Bus Selector4/8 -> Data Type Conversion44/1  "<VOUTP_LRRawWhlSpeedVTimeOut_flg>"
  Data Type Conversion92/1 -> R_HALOUT_APS_CSOP_ApsSetTimeout/60
  Bus Selector4/37 -> Data Type Conversion69/1  "<VOUTP_LongAccelVTimeOut_flg>"
  Data Type Conversion82/1 -> R_HALOUT_APS_CSOP_ApsSetTimeout/47
  Bus Selector4/39 -> Data Type Conversion71/1  "<VOUTP_BrkSwStaTimeOut_flg>"
  Ground_20/1 -> Data Type Conversion112/1
  Data Type Conversion75/1 -> R_HALOUT_APS_CSOP_ApsSetTimeout/33
  Bus Selector4/18 -> Data Type Conversion54/1  "<VOUTP_LFPulseCountTimeOut_flg>"
  Data Type Conversion74/1 -> R_HALOUT_APS_CSOP_ApsSetTimeout/38
  Bus Selector4/21 -> Data Type Conversion53/1  "<VOUTP_RRPulseCountTimeOut_flg>"
  Data Type Conversion58/1 -> R_HALOUT_APS_CSOP_ApsSetTimeout/25
  Data Type Conversion106/1 -> R_HALOUT_APS_CSOP_ApsSetTimeout/57
  Bus Selector4/24 -> Data Type Conversion57/1  "<VOUTP_EPSAOIControlTimeOut_flg>"
  Unit Delay3/1 -> [VHAL_NetworkReqCalled_flg]
  R_HALOUTCDD_CSOP_AppNmStateReq/1(Outport) -> Unit Delay3/1
  Ground/1 -> R_HALOUTCDD_CSOP_SleepRequest/1(SleepState)
  [BOUTP_outputs] -> Bus Selector/1
  Bus Selector/1 -> R_UDSCDD_CSOP_DdmRestartOperationCycle/Enable  "<VOUTP_EnterNewOperCyc_flg>"
  [BOUTP_outputs] -> Bus Selector1/1
  Bus Selector1/1 -> R_HALOUTCDD_CSOP_SetAcoreRebootCmdACK/Enable  "<VOUTP_AcoreRebootCmdACK_flg>"
  [BOUTP_outputs] -> Bus Selector5/1
  [BOUTP_outputs] -> Bus Selector2/1
  Real_DetectChange/1 -> R_HALIN_IMU_CSOP_IMUSetSta/Enable
  Bus Selector5/1 -> Real_DetectChange/1  "<VOUTP_IMUEnaCmd_flg>"
  Data Type Conversion97/1 -> R_HALIN_IMU_CSOP_IMUSetSta/1(u8_IMUEnaCmd)
  Bus Selector2/1 -> Data Type Conversion97/1  "<VOUTP_IMUEnaCmd_flg>"
  [BOUTP_outputs] -> Bus Selector7/1
  [BOUTP_DIDSetData_outputs] -> Bus Selector6/1
  Data Type Conversion107/1 -> Subsystem/1(In1)
  Bus Selector7/1 -> Subsystem/Enable  "<VOUTP_TPMSSensorIDRegStart_flg>"
  Bus Selector6/1 -> Data Type Conversion107/1  "<VHAL_TPMSSensorIDRegResults_raw8>"
  Bus Selector8/1 -> Detect Increase1/1  "<VOUTP_ResetPedalZeroPosStart_flg>"
  Detect Increase1/1 -> Subsystem1/Enable
  [BOUTP_outputs] -> Bus Selector8/1
  Function-Call Subsystem/1(u8Array256_NvmReadArrayInit) -> [u8Array256_NvmReadArrayInit]
  [u8Array256_NvmReadArray] -> Function-Call Subsystem/1(u8Array256_NvmReadArray)
  [trig_Read_NVM_AFTER_00] -> Function-Call Subsystem/Trigger
  [u8_AnyNMID] -> Latch/1
  Latch/1 -> Display/1  "VHAL_AnyNMIDLatch_flg"
  Constant7/1 -> Halin_CDD/25(u8_GetHWIDSta)
  [u8Array8_DidDataDKC] -> Halin_CDD/38(VHAL_GetDIDVCUKey_enum)
  [f32_GetAPS_DecReq] -> Halin_CDD/73(f32_GetAPS_DecReq)
  [u8_PwrReqOTA] -> Halin_CDD/30(VHAL_PwrReq_OTA_enum)
  [u8_ApsInSysFailSta] -> Halin_CDD/7(StaFSyaIn)
  [u8_DrDoorSW] -> Halin_CDD/14(VHAL_DrDoorSW_flg)
  [u8_RLDoorSW] -> Halin_CDD/17(VHAL_RLDoorSW_flg)
  [u8_HazardSW] -> Halin_CDD/19(VHAL_HazardSW_flg)
  [u8_RRDoorSW] -> Halin_CDD/16(VHAL_RRDoorSW_flg)
  Halin_CDD/4(BHAL_TPMS_outputs) -> [BHAL_TPMS_outputs]
  [u8_GetAPS_HW_Ver] -> Halin_CDD/66(u8_GetAPS_HW_Ver)
  [u8_GetAPS_Sta_System] -> Halin_CDD/69(u8_GetAPS_Sta_System)
  [u8_ClearDTCcmd] -> Halin_CDD/43(VHAL_ClearDTCcmd_flg)
  [u8_GetAPS_SW_Ver] -> Halin_CDD/65(u8_GetAPS_SW_Ver)
  [u8Array8_ApsInLevel] -> Halin_CDD/3(APSLevelData)
  [u16_AuxBattVol100mV] -> Halin_CDD/49(VHAL_AuxBattVolmV_100mV)
  Halin_CDD/5(BHAL_SYSTPMS_outputs) -> [BHAL_SYSTPMS_outputs]
  [BHAL_CAN4_outputs] -> Halin_CDD/42(BHAL_CAN4_outputs)
  [u8_GetCAAS_VMC_Req_A] -> Halin_CDD/79(u8_GetCAAS_VMC_Req_A)
  [u8_ResetPedalZeroPosReq] -> Halin_CDD/81(u8_ResetPedalZeroPosReq)
  [u8_TPMSDataInSta] -> Halin_CDD/39(TPMS_DataIn_flg)
  [f32_GetAPS_Angle_Target] -> Halin_CDD/68(f32_GetAPS_Angle_Target)
  [u8_GetAPS_Req] -> Halin_CDD/72(u8_GetAPS_Req)
  [u8_CrashSignal] -> Halin_CDD/23(VHAL_CrashSignalGPIO_flg)
  Halin_CDD/6(BHAL_DDM_outputs) -> [BHAL_DDM_outputs]
  [u8_GetAPS_ShftPosnReq] -> Halin_CDD/76(u8_GetAPS_ShftPosnReq)
  [u8_BrakeSW] -> Halin_CDD/11(VHAL_BrakeSWGPIO_flg)
  [u16_Pedal2Vol] -> Halin_CDD/10(VHAL_AccelPedal2Vol_Raw)
  [u8_AcoreRebootCmd] -> Halin_CDD/56(VHAL_AcoreRebootCmd_raw)
  [u8Array8_PasInDist] -> Halin_CDD/1(PASDistanceData)
  [u8Array12_ApsInUssSta] -> Halin_CDD/4(APSFaultStaData)
  [u8_IMUSixAxisValSta] -> Halin_CDD/47(VHAL_IMUSixAxisValSta_flg)
  Halin_CDD/7(BHAL_IMU_outputs) -> [BHAL_IMU_outputs]
  [BHAL_DID_outputs] -> Halin_CDD/55(BHAL_DIDGetData_raw)
  Halin_CDD/2(BHAL_GPIO_outputs) -> [BHAL_GPIO_outputs]
  Halin_CDD/3(BHAL_SYS_outputs) -> [BHAL_SYS_outputs]
  [u16_Pedal1Ref5V] -> Halin_CDD/50(VHAL_Pedal1Ref5V_raw)
  [u8_GetCAAS_Sta] -> Halin_CDD/78(u8_GetCAAS_Sta)
  [u8_ApsInSensorLayout] -> Halin_CDD/6(SNSRLayoutIn)
  [u8_CAN5BusOff] -> Halin_CDD/61(VHAL_CAN5BusOff_raw)
  [u8Array33_SWID] -> Halin_CDD/27(GetSWID_data)
  [u8_DidDataXWD] -> Halin_CDD/35(VHAL_DidXWDData_enum)
  [u8_TPMSSensorIDRegSta] -> Halin_CDD/80(u8_TPMSSensorIDRegSta)
  [u8_BootReason] -> Halin_CDD/53(VHAL_PmicBootReason_enum)
  Halin_CDD/1(BHAL_APM_outputs) -> [BHAL_APM_outputs]
  [u8_EvccAplusPwrUpReq] -> Halin_CDD/32(VHAL_EvccAplusPwrUpReq_flg)
  [u8_PsDoorSW] -> Halin_CDD/15(VHAL_PsDoorSW_flg)
  [u16_Pedal2Ref5V] -> Halin_CDD/51(VHAL_Pedal2Ref5V_raw)
  [s16_IMUSixAxisVal] -> Halin_CDD/45(VHAL_IMUSixAxisVal_raw)
  [u8_GetAPS_RQ_Display] -> Halin_CDD/64(u8_GetAPS_RQ_Display)
  [s8_AcoreReadyToSleep] -> Halin_CDD/33(VHAL_AcoreReadyToSlp_flg)
  [u8_GetAPS_Rq_EPAS_Ctrl] -> Halin_CDD/71(u8_GetAPS_Rq_EPAS_Ctrl)
  [f32_GetAPS_SpeedCmd] -> Halin_CDD/75(f32_GetAPS_SpeedCmd)
  [u8_ApsInSysMode] -> Halin_CDD/8(ModOperationIn)
  [u8Array9_TPMSData] -> Halin_CDD/40(TPMS_RawData)
  [u8_AllowMovThdOTA] -> Halin_CDD/31(VHAL_AllowMovThd_OTA_enum)
  [u8_GetAPS_VMC_Req_A] -> Halin_CDD/77(u8_GetAPS_VMC_Req_A)
  [u8_DidStaXWD] -> Halin_CDD/34(VHAL_DidXWDSta_flg)
  [u8_CurrentNMState] -> Halin_CDD/29(VHAL_CurrentNmState_enum)
  [u8_IMUOffsetValSta] -> Halin_CDD/46(VHAL_IMUOffsetValSta_flg)
  [u8Array256_NvmReadArrayInit] -> Halin_CDD/36(HAL_NvmReadData_raw)
  [u8_CAN4BusOff] -> Halin_CDD/60(VHAL_CAN4BusOff_raw)
  [u8_TailgateSW] -> Halin_CDD/13(VHAL_TailgateSW_flg)
  [trig_HAL_CDD_10_1] -> Halin_CDD/Trigger
  [u16_Pedal1Vol] -> Halin_CDD/9(VHAL_AccelPedal1Vol_Raw)
  Constant6/1 -> Halin_CDD/26(GetSWID_status)
  [u8_BrakeLamp] -> Halin_CDD/20(VHAL_BrakeLampSW_flg)
  [u8_GetAPS_ExitCondition] -> Halin_CDD/67(u8_GetAPS_ExitCondition)
  [u8_CTDSW] -> Halin_CDD/18(VHAL_CentralDoorLockSW_flg)
  [u32_WISR] -> Halin_CDD/54(VHAL_WisrBootReason_raw32)
  [u8_NvmProtectSta] -> Halin_CDD/48(VHAL_NvmProtectSta_flg)
  [s16_IMUOffsetVal] -> Halin_CDD/44(VHAL_IMUOffsetVal_raw)
  [BHAL_CAN2_outputs] -> Halin_CDD/41(BHAL_CAN2_outputs)
  [u8_CAN1BusOff] -> Halin_CDD/57(VHAL_CAN1BusOff_raw)
  [u8Array4_HWID] -> Halin_CDD/24(u8_HWID_4byte)
  [u8_AnyNMID] -> Halin_CDD/28(VHAL_AnyNMID_flg)
  [u8_GetAPS_DecReq_A] -> Halin_CDD/74(u8_GetAPS_DecReq_A)
  [u16Array4_ApsInDist] -> Halin_CDD/2(APSDistanceData)
  [VHAL_NetworkReqCalled_flg] -> Halin_CDD/52(VHAL_NetworkReqCalled_flg)
  [u8_GetAPS_Progress_PCT] -> Halin_CDD/63(u8_GetAPS_Progress_PCT)
  [u8_SeatSW] -> Halin_CDD/22(VHAL_SeatSW_flg)
  [u8_CAN3BusOff] -> Halin_CDD/59(VHAL_CAN3BusOff_raw)
  [u8_GetAPS_V_Rq_EPAS_Ctrl] -> Halin_CDD/70(u8_GetAPS_V_Rq_EPAS_Ctrl)
  [u8_CAN2BusOff] -> Halin_CDD/58(VHAL_CAN2BusOff_raw)
  [u8_DidStaDKC] -> Halin_CDD/37(VHAL_DIDVCUKeyReadSta_flg)
  [u8_TrunkHanSW] -> Halin_CDD/21(VHAL_TrunkHanSW_flg)
  [u8_HoodSW] -> Halin_CDD/12(VHAL_HoodSW_flg)
  [u8_ApsInPASChime] -> Halin_CDD/5(ChimeIn)
  Halin_CDD/8(Enable_decrypt) -> [Enable_decrypt]
  Halin_CDD/9(AESKey) -> Subsystem3/1(AESKey)
  Halin_CDD/10(DKCRawData) -> Subsystem3/2(DKCRawData)
  [trig_HAL_DKC_10_2] -> Subsystem3/Trigger
  Subsystem3/1(u8Array16_ResultData) -> [u8Array16_ResultData]
  [Enable_decrypt] -> Subsystem4/1(Enable_Decrypt)
  [trig_HAL_DKC_10_3] -> Subsystem4/Trigger
  [u8Array16_ResultData] -> Subsystem4/2(u8Array16_ResultData)
  Subsystem4/1(BHAL_DKC_outputs) -> [BHAL_DKC_outputs]
  [BHAL_SYS_outputs] -> OUTP_AFTER/3(BHAL_SYS_outputs)
  OUTP_AFTER/7(HAL_NvmWriteData_raw) -> [u8Array256_NvmWriteArray]
  OUTP_AFTER/5(ApsOut_SetVehSpdTOCmd) -> [u8_ApsOutSetVehSpdTOCmd]
  OUTP_AFTER/12(BOUTP_DIDSetData_outputs) -> [BOUTP_DIDSetData_outputs]
  OUTP_AFTER/1(ApsOut_GearPosnSig) -> [u8_ApsOutGearPosnSig]
  OUTP_AFTER/3(ApsOut_SetFrSensorOnCmd) -> [u8_ApsOutSetFrSensorOnCmd]
  OUTP_AFTER/2(ApsOut_SendChrgPlugStaSig) -> [u8_ApsOutSendChrgPlugSta]
  [u8Array256_NvmReadArray] -> OUTP_AFTER/4(VHAL_NvmReadArray_raw)
  OUTP_AFTER/8(DTC_Trigger) -> [DTC_Trigger]
  [trig_OUTP_AFTER_40_1] -> OUTP_AFTER/Trigger
  OUTP_AFTER/11(DTC_Array) -> [DTC_Array]
  OUTP_AFTER/6(ApsOut_VehSpdSig) -> [f32_ApsOutVehSpdSig]
  [BHAL_SYSTPMS_outputs] -> OUTP_AFTER/2(BHAL_SYSTPMS_outputs)
  [BOUTP_outputs] -> OUTP_AFTER/1(BOUTP_outputs)
  OUTP_AFTER/4(ApsOut_SetFrSensorSwTOCmd) -> [u8_ApsOutSetFrSensorSwTOCmd]
  OUTP_AFTER/9(Header_Array) -> [Header_Array]
  R_HALINCDD_CSOP_ResetPedalZeroPosReq/1 -> [u8_ResetPedalZeroPosReq]
  R_HALINCDD_CSOP_TPMSSensorIDRegGetSta/1 -> [u8_TPMSSensorIDRegSta]
  R_HALINCDD_CSOP_ReadPedalZeroPosReq/1 -> [u8_ReadPedalZeroPosReq]
  hcu_main_sched/1(trig_Read_NVM_00()) -> [trig_Read_NVM_00]
  hcu_main_sched/8(trig_HAL_DKC_10_2()) -> [trig_HAL_DKC_10_2]
  hcu_main_sched/3(trig_WDG()) -> [trig_WDG]
  hcu_main_sched/15(trig_HAL_OUTAFTER_50_1()) -> [trig_HAL_OUTAFTER_50_1]
  hcu_main_sched/6(trig_HAL_IN_10()) -> [trig_HAL_IN_10]
  hcu_main_sched/5(trig_GetDID()) -> [trig_GetDID]
  hcu_main_sched/14(trig_HAL_OUT_50()) -> [trig_HAL_OUT_50]
  Detect Increase/1 -> hcu_main_sched/2(VHAL_ChkNVM_flg)  "VHAL_ChkNVM_flg"
  hcu_main_sched/12(trig_OUTP_40()) -> [trig_OUTP_40]
  Constant5/1 -> hcu_main_sched/1(VHAL_FusionSchedReq_flg)
  [u8_ReadPedalZeroPosReq] -> Detect Increase/1
  hcu_main_sched/16(trig_Read_NVM_AFTER_00()) -> [trig_Read_NVM_AFTER_00]
  hcu_main_sched/9(trig_HAL_DKC_10_3()) -> [trig_HAL_DKC_10_3]
  hcu_main_sched/11(trig_APP_30()) -> [trig_APP_30]
  hcu_main_sched/4(trig_GetNMID()) -> [trig_GetNMID]
  hcu_main_sched/13(trig_OUTP_AFTER_40_1()) -> [trig_OUTP_AFTER_40_1]
  hcu_main_sched/7(trig_HAL_CDD_10_1()) -> [trig_HAL_CDD_10_1]
  hcu_main_sched/2(trig_ReadIMUOffset_00()) -> [trig_ReadIMUOffset_00]
  hcu_main_sched/10(trig_INP_20()) -> [trig_INP_20]
  INP/3 -> [BINP_CAN3_outputs], APP/3
  [BHAL_SYS_outputs] -> INP/9
  INP/1 -> [BINP_CAN1_outputs], APP/1
  [s8_AcoreReadyToSleep] -> HAL_OUT/3
  [BHAL_GPIO_outputs] -> INP/7
  [BHAL_APM_outputs] -> INP/10
  HAL_IN/3 -> INP/3
  [BHAL_IMU_outputs] -> INP/13
  [trig_APP_30] -> APP/Trigger
  [trig_INP_20] -> INP/Trigger
  INP/13 -> APP/13
  [trig_HAL_IN_10] -> HAL_IN/Trigger
  [BHAL_DDM_outputs] -> INP/12
  [BHAL_DKC_outputs] -> INP/11
  HAL_IN/2 -> [BHAL_CAN2_outputs], INP/2
  INP/5 -> [BINP_CAN5_outputs], APP/5
  HAL_IN/1 -> INP/1
  INP/9 -> APP/9
  HAL_IN/5 -> INP/5
  OUTP/1 -> HAL_OUT/1, [BOUTP_outputs]
  INP/12 -> APP/12
  INP/6 -> [BINP_CAN6_outputs], APP/6
  HAL_IN/6 -> INP/6
  [trig_OUTP_40] -> OUTP/Trigger
  INP/7 -> APP/7
  HAL_IN/4 -> [BHAL_CAN4_outputs], INP/4
  INP/11 -> APP/11
  [BHAL_TPMS_outputs] -> INP/8
  INP/10 -> [BINP_APM_outputs], APP/10
  INP/4 -> [BINP_CAN4_outputs], APP/4
  INP/2 -> [BINP_CAN2_outputs], APP/2
  [trig_HAL_OUT_50] -> HAL_OUT/Trigger
  INP/8 -> APP/8
  [u8_GetRAPS_ErrLv1_flg] -> Halin_CDD/86(u8_GetRAPS_ErrLv1_flg)
  [u8_GetAPS_PwrReq_cmd] -> Halin_CDD/82(u8_GetAPS_PwrReq_cmd)
  [u8_GetRAPS_BCM_LockReq_Cmd] -> Halin_CDD/83(u8_GetRAPS_BCM_LockReq_Cmd)
  [u8_GetRAPS_BCM_Lamp_Cmd] -> Halin_CDD/84(u8_GetRAPS_BCM_Lamp_Cmd)
  [u8_GetRAPS_ErrWarn_Sta] -> Halin_CDD/85(u8_GetRAPS_ErrWarn_Sta)
  R_CAN1_ABM1_CAN1_SG_ABM1_read/1 -> HAL_IN/1
  R_CAN1_EPB1_CAN1_SG_EPB1_read/1 -> HAL_IN/2
  R_CAN1_EPS1_CAN1_SG_EPS1_read/1 -> HAL_IN/3
  R_CAN1_ESC1_CAN1_SG_ESC1_read/1 -> HAL_IN/4
  R_CAN1_ESC5_CAN1_SG_ESC5_read/1 -> HAL_IN/5
  R_CAN1_eBST1_CAN1_SG_eBST1_read/1 -> HAL_IN/6
  R_CAN2_HMI1_CAN2_SG_HMI1_read/1 -> HAL_IN/7
  R_CAN2_IVI1_CAN2_SG_IVI1_read/1 -> HAL_IN/8
  R_CAN2_IVI2_CAN2_SG_IVI2_read/1 -> HAL_IN/9
  R_CAN2_IVI3_CAN2_SG_IVI3_read/1 -> HAL_IN/10
  R_CAN2_METER1_CAN2_SG_METER1_read/1 -> HAL_IN/11
  R_CAN3_BMS1_CAN3_SG_BMS1_read/1 -> HAL_IN/12
  R_CAN3_BMS3_CAN3_SG_BMS3_read/1 -> HAL_IN/13
  R_CAN3_BMS4_CAN3_SG_BMS4_read/1 -> HAL_IN/14
  R_CAN3_BMS5_CAN3_SG_BMS5_read/1 -> HAL_IN/15
  R_CAN3_BMS6_CAN3_SG_BMS6_read/1 -> HAL_IN/16
  R_CAN3_BMS8_CAN3_SG_BMS8_read/1 -> HAL_IN/17
  R_CAN3_CCU1_CAN3_SG_CCU1_read/1 -> HAL_IN/18
  R_CAN3_CCU2_CAN3_SG_CCU2_read/1 -> HAL_IN/19
  R_CAN3_EBM1_CAN3_SG_EBM1_read/1 -> HAL_IN/20
  R_CAN3_MCU_B_F1_CAN3_SG_MCU_B_F1_read/1 -> HAL_IN/21
  R_CAN3_MCU_B_F2_CAN3_SG_MCU_B_F2_read/1 -> HAL_IN/22
  R_CAN3_MCU_B_R1_CAN3_SG_MCU_B_R1_read/1 -> HAL_IN/23
  R_CAN3_MCU_B_R2_CAN3_SG_MCU_B_R2_read/1 -> HAL_IN/24
  R_CAN3_MCU_N_F1_CAN3_SG_MCU_N_F1_read/1 -> HAL_IN/25
  R_CAN3_MCU_N_F2_CAN3_SG_MCU_N_F2_read/1 -> HAL_IN/26
  R_CAN3_MCU_N_F3_CAN3_SG_MCU_N_F3_read/1 -> HAL_IN/27
  R_CAN3_MCU_N_R1_CAN3_SG_MCU_N_R1_read/1 -> HAL_IN/28
  R_CAN3_MCU_N_R2_CAN3_SG_MCU_N_R2_read/1 -> HAL_IN/29
  R_CAN3_MCU_N_R3_CAN3_SG_MCU_N_R3_read/1 -> HAL_IN/30
  R_CAN3_Shifter1_CAN3_SG_Shifter1_read/1 -> HAL_IN/31
  R_CAN3_Shifter2_CAN3_SG_Shifter2_read/1 -> HAL_IN/32
  R_CAN4_BodyZone_DR1_CAN4_SG_BodyZone_DR1_read/1 -> HAL_IN/33
  HAL_OUT/1 -> P_CAN1_FD1_BCM1_CAN1_SG_FD1_BCM1_write/1
  HAL_OUT/2 -> P_CAN1_FD1_VCU1_CAN1_SG_FD1_VCU1_write/1
  HAL_OUT/3 -> P_CAN1_FD1_VMC1_CAN1_SG_FD1_VMC1_write/1
  HAL_OUT/4 -> P_CAN2_FD2_CE100_0_CAN2_SG_FD2_CE100_0_write/1
  HAL_OUT/5 -> P_CAN2_FD2_CE200_1_CAN2_SG_FD2_CE200_1_write/1
  HAL_OUT/6 -> P_CAN2_GW2_CE100_0_CAN2_SG_GW2_CE100_0_write/1
  HAL_OUT/7 -> P_CAN2_GW2_CE200_0_CAN2_SG_GW2_CE200_0_write/1
  HAL_OUT/8 -> P_CAN3_FD3_BCM1_CAN3_SG_FD3_BCM1_write/1
  HAL_OUT/9 -> P_CAN3_FD3_THCM2_CAN3_SG_FD3_THCM2_write/1
  HAL_OUT/10 -> P_CAN3_FD3_V2L1_CAN3_SG_FD3_V2L1_write/1
  HAL_OUT/11 -> P_CAN4_FD4_CE100_1_CAN4_SG_FD4_CE100_1_write/1
  HAL_OUT/12 -> P_CAN4_FD4_CE200_0_CAN4_SG_FD4_CE200_0_write/1
  HAL_OUT/13 -> P_CAN4_GW4_CE100_0_CAN4_SG_GW4_CE100_0_write/1
  HAL_OUT/14 -> P_CAN5_FD5_CE100_0_CAN5_SG_FD5_CE100_0_write/1
  HAL_OUT/15 -> P_CAN5_FD5_Debug1_CAN5_SG_FD5_Debug1_write/1
  HAL_OUT/16 -> P_CAN5_FD5_Debug2_CAN5_SG_FD5_Debug2_write/1
  HAL_OUT/17 -> P_CAN6_FD6_BCM1_CAN6_SG_FD6_BCM1_write/1
  HAL_OUT/18 -> P_CAN6_FD6_VCU1_CAN6_SG_FD6_VCU1_write/1
  HAL_OUT/19 -> P_CAN6_FD6_VMC1_CAN6_SG_FD6_VMC1_write/1
  HAL_OUT/20 -> P_CAN6_GW6_CE100_0_CAN6_SG_GW6_CE100_0_write/1
  HAL_OUT/21 -> IRV_ms10_CAN1_SG_FD1_APS3_write/1
  HAL_OUT/22 -> IRV_ms10_CAN1_SG_FD1_VCU2_write/1
  HAL_OUT/23 -> IRV_ms10_CAN1_SG_FD1_VCU3_write/1
  HAL_OUT/24 -> IRV_ms10_CAN1_SG_VMC_FCM1_write/1
  HAL_OUT/25 -> IRV_ms10_CAN3_SG_FD3_VCU0_write/1
  HAL_OUT/26 -> IRV_ms10_CAN3_SG_FD3_VCU2_write/1
  HAL_OUT/27 -> IRV_ms10_CAN3_SG_FD3_VCU2_toNIDEC_write/1
  HAL_OUT/28 -> IRV_ms10_CAN3_SG_FD3_VCU5_write/1
  HAL_OUT/29 -> IRV_ms10_CAN3_SG_GW_ESC1_toNIDEC_write/1
  HAL_OUT/30 -> IRV_ms10_CAN5_SG_FD5_Debug3_write/1
  HAL_OUT/31 -> IRV_ms10_CAN6_SG_FD6_APS3_write/1
  HAL_OUT/32 -> IRV_ms10_CAN6_SG_FD6_VCU2_write/1
  HAL_OUT/33 -> IRV_ms100_CAN1_SG_FD1_THCM1_write/1
  HAL_OUT/34 -> IRV_ms100_CAN3_SG_FD3_THCM1_write/1
  HAL_OUT/35 -> IRV_ms1000_CAN3_SG_GW_IVI6_toNIDEC_write/1
  HAL_OUT/36 -> IRV_ms20_CAN1_SG_FD1_APS2_write/1
  HAL_OUT/37 -> IRV_ms20_CAN2_SG_FD2_C20_0_write/1
  HAL_OUT/38 -> IRV_ms500_CAN1_SG_FD1_VMC2_write/1
  HAL_OUT/39 -> IRV_ms5000_CAN2_SG_FD2_Version_write/1
  HAL_OUT/40 -> IRV_E2E_CAN3_SG_FD3_VCU1_write/1
  HAL_OUT/41 -> IRV_E2E_CAN3_SG_FD3_VCU1_toNIDEC_write/1
  HAL_OUT/42 -> IRV_E2E_CAN4_SG_FD4_CE100_0_write/1
  HAL_OUT/43 -> [E2E_CAN3_VCU1_Trigger]
  HAL_OUT/44 -> [E2E_CAN3_VCU1_toNIDEC_Trigger]
  HAL_OUT/45 -> [E2E_CAN4_VCU1_Trigger]
  Data Type Conversion/1 -> Subsystem5/1(In1)
  detect_change1/1 -> Subsystem5/Enable
  R_UDSCDD_CSOP_SetDTCStatus/1(retSta) -> Terminator_11/1
  [BHAL_DID_outputs] -> OUTP_AFTER/5(BHAL_DIDGetData_raw)
  [BOUTP_outputs] -> Bus Selector10/1
  [BOUTP_outputs] -> Bus Selector11/1
  [BOUTP_outputs] -> Bus Selector12/1
  [BOUTP_outputs] -> Bus Selector13/1
  [BOUTP_outputs] -> Bus Selector14/1
  [BOUTP_outputs] -> Bus Selector15/1
  [BOUTP_outputs] -> Bus Selector16/1
  [BOUTP_outputs] -> Bus Selector17/1
  Constant8/1 -> Subsystem6/Enable
  Subsystem6/1(u8Array17_VinCode) -> Subsystem7/1(u8Array17_VinCode)
  Data Type Conversion119/1 -> R_HALOUT_APS_CSOP_ApsSetData/83
  Data Type Conversion26/1 -> R_HALOUT_APS_CSOP_ApsSetData/41
  Data Type Conversion118/1 -> R_HALOUT_APS_CSOP_ApsSetData/82
  Bus Selector3/16 -> Data Type Conversion10/1  "<VOUTP_LFPulseCountV_flg>"
  Bus Selector3/44 -> Data Type Conversion29/1  "<VOUTP_BrkSwV_flg>"
  Bus Selector3/60 -> R_HALOUT_APS_CSOP_ApsSetData/60  "<VOUTP_IVIScreen_enum>"
  Bus Selector3/22 -> Data Type Conversion15/1  "<VOUTP_LRPulseCount_enum>"
  Bus Selector3/35 -> R_HALOUT_APS_CSOP_ApsSetData/35  "<VOUTP_YawRate_degps>"
  Bus Selector3/6 -> R_HALOUT_APS_CSOP_ApsSetData/6  "<VOUTP_LRRawWhlSpeed_kph>"
  Bus Selector3/70 -> R_HALOUT_APS_CSOP_ApsSetData/70  "<VOUTP_LFPressIndi_enum>"
  Bus Selector3/2 -> R_HALOUT_APS_CSOP_ApsSetData/2  "<VOUTP_BrkPedalPos_pct>"
  Data Type Conversion35/1 -> R_HALOUT_APS_CSOP_ApsSetData/53
  Bus Selector3/53 -> Data Type Conversion35/1  "<VOUTP_TailgateSW_flg>"
  Data Type Conversion102/1 -> R_HALOUT_APS_CSOP_ApsSetData/64
  Data Type Conversion99/1 -> R_HALOUT_APS_CSOP_ApsSetData/9
  Bus Selector3/58 -> Data Type Conversion37/1  "<VOUTP_IVIStatus_flg>"
  Bus Selector3/23 -> Data Type Conversion16/1  "<VOUTP_RRPulseCount_enum>"
  Data Type Conversion13/1 -> R_HALOUT_APS_CSOP_ApsSetData/19
  Bus Selector3/59 -> R_HALOUT_APS_CSOP_ApsSetData/59  "<VOUTP_CAASSw_enum>"
  Data Type Conversion30/1 -> R_HALOUT_APS_CSOP_ApsSetData/45
  Bus Selector3/61 -> Data Type Conversion105/1  "<VOUTP_CAASCtrlAvail_flg>"
  Bus Selector3/56 -> R_HALOUT_APS_CSOP_ApsSetData/56  "<VOUTP_AVMParkingmode_enum>"
  Data Type Conversion14/1 -> R_HALOUT_APS_CSOP_ApsSetData/21
  Bus Selector3/25 -> Data Type Conversion18/1  "<VOUTP_APSCtrlAvail_flg>"
  Data Type Conversion29/1 -> R_HALOUT_APS_CSOP_ApsSetData/44
  Data Type Conversion105/1 -> R_HALOUT_APS_CSOP_ApsSetData/61
  Bus Selector3/62 -> Data Type Conversion104/1  "<VOUTP_ABSActive_flg>"
  Bus Selector3/9 -> Data Type Conversion99/1  "<VOUTP_RFRawWhlSpeedV_flg>"
  Data Type Conversion15/1 -> R_HALOUT_APS_CSOP_ApsSetData/22
  Bus Selector3/27 -> R_HALOUT_APS_CSOP_ApsSetData/27  "<VOUTP_DriIntend_enum>"
  Data Type Conversion10/1 -> R_HALOUT_APS_CSOP_ApsSetData/16
  Data Type Conversion37/1 -> R_HALOUT_APS_CSOP_ApsSetData/58
  Bus Selector3/34 -> R_HALOUT_APS_CSOP_ApsSetData/34  "<VOUTP_GRADE_Deg>"
  Bus Selector3/48 -> Data Type Conversion32/1  "<VOUTP_EPBExtApplyAvail_flg>"
  Data Type Conversion27/1 -> R_HALOUT_APS_CSOP_ApsSetData/42
  Data Type Conversion23/1 -> R_HALOUT_APS_CSOP_ApsSetData/33
  Bus Selector3/43 -> Data Type Conversion28/1  "<VOUTP_BrkSwSta_flg>"
  Bus Selector3/14 -> R_HALOUT_APS_CSOP_ApsSetData/14  "<VOUTP_LRWhlRotDir_enum>"
  Data Type Conversion20/1 -> R_HALOUT_APS_CSOP_ApsSetData/20
  Bus Selector3/64 -> Data Type Conversion102/1  "<VOUTP_DriverSeatBeltCmd_flg>"
  Data Type Conversion125/1 -> R_HALOUT_APS_CSOP_ApsSetData/67
  Bus Selector3/51 -> Data Type Conversion33/1  "<VOUTP_AllDoorSW_flg>"
  [BOUTP_outputs] -> Bus Selector3/1
  Bus Selector3/66 -> Data Type Conversion100/1  "<VOUTP_PsDoorSW_flg>"
  Bus Selector3/8 -> Data Type Conversion98/1  "<VOUTP_LFRawWhlSpeedV_flg>"
  Data Type Conversion33/1 -> R_HALOUT_APS_CSOP_ApsSetData/51
  Data Type Conversion12/1 -> R_HALOUT_APS_CSOP_ApsSetData/18
  Data Type Conversion22/1 -> R_HALOUT_APS_CSOP_ApsSetData/32
  Data Type Conversion36/1 -> R_HALOUT_APS_CSOP_ApsSetData/57
  Data Type Conversion25/1 -> R_HALOUT_APS_CSOP_ApsSetData/40
  Bus Selector3/55 -> R_HALOUT_APS_CSOP_ApsSetData/55  "<VOUTP_AVMparkingexcute_enum>"
  Bus Selector3/63 -> Data Type Conversion103/1  "<VOUTP_TCSActive_flg>"
  Bus Selector3/45 -> Data Type Conversion30/1  "<VOUTP_ESCStandstill_flg>"
  Bus Selector3/75 -> Data Type Conversion122/1  "<VOUTP_CAASActive_flg>"
  Bus Selector3/1 -> R_HALOUT_APS_CSOP_ApsSetData/1  "<VOUTP_PowerSta_enum>"
  Data Type Conversion121/1 -> R_HALOUT_APS_CSOP_ApsSetData/11
  Bus Selector3/50 -> R_HALOUT_APS_CSOP_ApsSetData/50  "<VOUTP_EPBSta_enum>"
  Bus Selector3/13 -> R_HALOUT_APS_CSOP_ApsSetData/13  "<VOUTP_RFWhlRotDir_enum>"
  Bus Selector3/33 -> Data Type Conversion23/1  "<VOUTP_SASV_flg>"
  Data Type Conversion120/1 -> R_HALOUT_APS_CSOP_ApsSetData/10
  Data Type Conversion24/1 -> R_HALOUT_APS_CSOP_ApsSetData/39
  Bus Selector3/7 -> R_HALOUT_APS_CSOP_ApsSetData/7  "<VOUTP_RRRawWhlSpeed_kph>"
  Bus Selector3/73 -> R_HALOUT_APS_CSOP_ApsSetData/73  "<VOUTP_sigAmbAirT_C>"
  Bus Selector3/32 -> Data Type Conversion22/1  "<VOUTP_SASCAL_flg>"
  Bus Selector3/71 -> R_HALOUT_APS_CSOP_ApsSetData/71  "<VOUTP_RRPressIndi_enum>"
  Bus Selector3/37 -> R_HALOUT_APS_CSOP_ApsSetData/37  "<VOUTP_LongAccel_Gps>"
  Bus Selector3/30 -> R_HALOUT_APS_CSOP_ApsSetData/30  "<VOUTP_SASSpeed_degps>"
  Data Type Conversion28/1 -> R_HALOUT_APS_CSOP_ApsSetData/43
  Data Type Conversion18/1 -> R_HALOUT_APS_CSOP_ApsSetData/25
  Bus Selector3/42 -> Data Type Conversion27/1  "<VOUTP_MCPressureV_bar>"
  Bus Selector3/49 -> R_HALOUT_APS_CSOP_ApsSetData/49  "<VOUTP_EPBErrSta_enum>"
  Bus Selector3/24 -> Data Type Conversion17/1  "<VOUTP_APSActive_flg>"
  Bus Selector3/68 -> Data Type Conversion124/1  "<VOUTP_RRDoorSW_flg>"
  Bus Selector3/20 -> Data Type Conversion20/1  "<VOUTP_LFPulseCount_enum>"
  Data Type Conversion11/1 -> R_HALOUT_APS_CSOP_ApsSetData/17
  Bus Selector3/54 -> R_HALOUT_APS_CSOP_ApsSetData/54  "<VOUTP_AVMparkingcancel_enum>"
  Data Type Conversion100/1 -> R_HALOUT_APS_CSOP_ApsSetData/66
  Bus Selector3/26 -> R_HALOUT_APS_CSOP_ApsSetData/26  "<VOUTP_ShifterHandleCmd_enum>"
  Bus Selector3/40 -> Data Type Conversion25/1  "<VOUTP_LatAccelV_flg>"
  Bus Selector3/19 -> Data Type Conversion13/1  "<VOUTP_RRPulseCountV_flg>"
  Bus Selector3/76 -> Data Type Conversion5/1  "<VOUTP_PwrReqRAPSAvail_flg>"
  Bus Selector3/10 -> Data Type Conversion120/1  "<VOUTP_LRRawWhlSpeedV_flg>"
  Bus Selector3/15 -> R_HALOUT_APS_CSOP_ApsSetData/15  "<VOUTP_RRWhlRotDir_enum>"
  Bus Selector3/47 -> Data Type Conversion31/1  "<VOUTP_EPBExtReleaseAvail_flg>"
  Bus Selector3/21 -> Data Type Conversion14/1  "<VOUTP_RFPulseCount_enum>"
  Data Type Conversion98/1 -> R_HALOUT_APS_CSOP_ApsSetData/8
  Bus Selector3/39 -> Data Type Conversion24/1  "<VOUTP_YawRateV_flg>"
  Data Type Conversion103/1 -> R_HALOUT_APS_CSOP_ApsSetData/63
  Bus Selector3/12 -> R_HALOUT_APS_CSOP_ApsSetData/12  "<VOUTP_LFWhlRotDir_enum>"
  Bus Selector3/78 -> Data Type Conversion8/1  "<VOUTP_DKCParkingModeCmd_enum>"
  Bus Selector3/46 -> R_HALOUT_APS_CSOP_ApsSetData/46  "<VOUTP_ESCAPSSta_enum>"
  Data Type Conversion124/1 -> R_HALOUT_APS_CSOP_ApsSetData/68
  Bus Selector3/77 -> Data Type Conversion7/1  "<VOUTP_DKCPDkeyAreaRAPSSta_enum>"
  Data Type Conversion101/1 -> R_HALOUT_APS_CSOP_ApsSetData/65
  Bus Selector3/67 -> Data Type Conversion125/1  "<VOUTP_RLDoorSW_flg>"
  Bus Selector3/5 -> R_HALOUT_APS_CSOP_ApsSetData/5  "<VOUTP_RFRawWhlSpeed_kph>"
  Data Type Conversion104/1 -> R_HALOUT_APS_CSOP_ApsSetData/62
  Data Type Conversion34/1 -> R_HALOUT_APS_CSOP_ApsSetData/52
  Bus Selector3/65 -> Data Type Conversion101/1  "<VOUTP_DrDoorSW_flg>"
  Bus Selector3/29 -> R_HALOUT_APS_CSOP_ApsSetData/29  "<VOUTP_SASAngle_Deg>"
  Data Type Conversion32/1 -> R_HALOUT_APS_CSOP_ApsSetData/48
  Bus Selector3/28 -> R_HALOUT_APS_CSOP_ApsSetData/28  "<VOUTP_EPSAOIControl_enum>"
  Data Type Conversion96/1 -> R_HALOUT_APS_CSOP_ApsSetData/74
  Bus Selector3/80 -> Data Type Conversion9/1  "<VOUTP_DrSeatSta_enum>"
  Data Type Conversion7/1 -> R_HALOUT_APS_CSOP_ApsSetData/77
  Bus Selector3/31 -> Data Type Conversion21/1  "<VOUTP_SASSpeedValid_flg>"
  Data Type Conversion31/1 -> R_HALOUT_APS_CSOP_ApsSetData/47
  Data Type Conversion8/1 -> R_HALOUT_APS_CSOP_ApsSetData/78
  Bus Selector3/4 -> R_HALOUT_APS_CSOP_ApsSetData/4  "<VOUTP_LFRawWhlSpeed_kph>"
  Data Type Conversion6/1 -> R_HALOUT_APS_CSOP_ApsSetData/79
  Bus Selector3/36 -> R_HALOUT_APS_CSOP_ApsSetData/36  "<VOUTP_LatAccel_Gps>"
  Bus Selector3/18 -> Data Type Conversion12/1  "<VOUTP_LRPulseCountV_flg>"
  Data Type Conversion117/1 -> R_HALOUT_APS_CSOP_ApsSetData/81
  Bus Selector3/52 -> Data Type Conversion34/1  "<VOUTP_HoodSW_flg>"
  Data Type Conversion17/1 -> R_HALOUT_APS_CSOP_ApsSetData/24
  Data Type Conversion16/1 -> R_HALOUT_APS_CSOP_ApsSetData/23
  Data Type Conversion5/1 -> R_HALOUT_APS_CSOP_ApsSetData/76
  Bus Selector3/83 -> Data Type Conversion119/1  "<VOUTP_IVIUserTakeOverAPSSta_flg>"
  Bus Selector3/69 -> R_HALOUT_APS_CSOP_ApsSetData/69  "<VOUTP_RFPressIndi_enum>"
  Data Type Conversion21/1 -> R_HALOUT_APS_CSOP_ApsSetData/31
  Data Type Conversion122/1 -> R_HALOUT_APS_CSOP_ApsSetData/75
  Bus Selector3/57 -> Data Type Conversion36/1  "<VOUTP_AVMErrSTA_flg>"
  Bus Selector3/74 -> Data Type Conversion96/1  "<VOUTP_VehActSpd_kph>"
  Bus Selector3/82 -> Data Type Conversion118/1  "<VOUTP_VCURAPSErrLv3_flg>"
  Bus Selector3/3 -> R_HALOUT_APS_CSOP_ApsSetData/3  "<VOUTP_ActAPSPosn_pct>"
  Bus Selector3/11 -> Data Type Conversion121/1  "<VOUTP_RRRawWhlSpeedV_flg>"
  Bus Selector3/38 -> R_HALOUT_APS_CSOP_ApsSetData/38  "<VOUTP_MCPressure_bar>"
  Bus Selector3/81 -> Data Type Conversion117/1  "<VOUTP_VCURAPSErrLv2_flg>"
  Bus Selector3/72 -> R_HALOUT_APS_CSOP_ApsSetData/72  "<VOUTP_LRPressIndi_enum>"
  Bus Selector3/41 -> Data Type Conversion26/1  "<VOUTP_LongAccelV_flg>"
  Bus Selector3/79 -> Data Type Conversion6/1  "<VOUTP_PUIDLowPower_flg>"
  Data Type Conversion9/1 -> R_HALOUT_APS_CSOP_ApsSetData/80
  Bus Selector3/17 -> Data Type Conversion11/1  "<VOUTP_RFPulseCountV_flg>"
  R_HALINCDD_CSOP_CAN6BusOff/1 -> [u8_CAN6BusOff]
  [u8_CAN6BusOff] -> Halin_CDD/62(VHAL_CAN6BusOff_raw)
  R_HALINCDD_CSOP_GetBootPath/1 -> [u32_BootPath]
  [u32_BootPath] -> Halin_CDD/87(u32_BootPath)
  APP/9 -> OUTP/9
  APP/8 -> OUTP/8
  APP/10 -> OUTP/10
  APP/7 -> OUTP/7
  APP/11 -> OUTP/11
  APP/6 -> OUTP/6
  APP/12 -> OUTP/12
  APP/5 -> OUTP/5
  APP/13 -> OUTP/13
  APP/4 -> OUTP/4
  APP/14 -> OUTP/14
  APP/3 -> OUTP/3
  APP/15 -> OUTP/15
  APP/2 -> OUTP/2
  APP/16 -> OUTP/16
  APP/1 -> OUTP/1
  APP/17 -> HAL_OUT/2
  R_CAN4_BodyZone_PS1_CAN4_SG_BodyZone_PS1_read/1 -> HAL_IN/35
  R_CAN4_BodyZone_PS2_CAN4_SG_BodyZone_PS2_read/1 -> HAL_IN/36
  R_CAN4_DKC1_CAN4_SG_DKC1_read/1 -> HAL_IN/37
  R_CAN4_DKC2_CAN4_SG_DKC2_read/1 -> HAL_IN/38
  R_CAN4_PTG1_CAN4_SG_PTG1_read/1 -> HAL_IN/39
  R_CAN4_ZONE_DR1_CAN4_SG_ZONE_DR1_read/1 -> HAL_IN/40
  R_CAN4_ZONE_DR_VCU_CAN4_SG_ZONE_DR_VCU_read/1 -> HAL_IN/41
  R_CAN4_ZONE_FR1_CAN4_SG_ZONE_FR1_read/1 -> HAL_IN/42
  R_CAN4_ZONE_FR_VCU_CAN4_SG_ZONE_FR_VCU_read/1 -> HAL_IN/43
  R_CAN4_zGW_APTC1_CAN4_SG_zGW_APTC1_read/1 -> HAL_IN/44
  R_CAN4_zGW_CANFr1_CAN4_SG_zGW_CANFr1_read/1 -> HAL_IN/45
  R_CAN4_zGW_LINDr1_CAN4_SG_zGW_LINDr1_read/1 -> HAL_IN/46
  R_CAN4_zGW_LINDr2_CAN4_SG_zGW_LINDr2_read/1 -> HAL_IN/47
  R_CAN4_zGW_LINFr1_CAN4_SG_zGW_LINFr1_read/1 -> HAL_IN/48
  R_CAN4_zGW_LINFr2_CAN4_SG_zGW_LINFr2_read/1 -> HAL_IN/49
  R_CAN4_zGW_SEAT1_CAN4_SG_zGW_SEAT1_read/1 -> HAL_IN/50
  R_CAN6_FCM1_CAN6_SG_FCM1_read/1 -> HAL_IN/54
  R_CAN6_FCM2_CAN6_SG_FCM2_read/1 -> HAL_IN/55
  R_CAN6_FCM3_CAN6_SG_FCM3_read/1 -> HAL_IN/56
  R_CAN6_FCM4_CAN6_SG_FCM4_read/1 -> HAL_IN/57
  R_CAN6_SRR1_CAN6_SG_SRR1_read/1 -> HAL_IN/58
  R_CAN4_BodyZone_DR2_CAN4_SG_BodyZone_DR2_read/1 -> HAL_IN/34
  R_HALINCDD_CSOP_nmGetCan1RxErrorCount/1 -> [u8_pCan1RxErrorCount]
  Constant9/1 -> R_HALINCDD_CSOP_nmGetCan1RxErrorCount/2
  R_HALINCDD_CSOP_nmGetCan1TxErrorCount/1 -> [u8_pCan1TxErrorCount]
  Constant10/1 -> R_HALINCDD_CSOP_nmGetCan1TxErrorCount/2
  Constant11/1 -> R_HALINCDD_CSOP_nmGetCan1RxErrorCount/1
  Constant12/1 -> R_HALINCDD_CSOP_nmGetCan1TxErrorCount/1
  Constant16/1 -> R_HALINCDD_CSOP_nmGetCan2TxErrorCount/2
  Constant14/1 -> R_HALINCDD_CSOP_nmGetCan2RxErrorCount/1
  Constant15/1 -> R_HALINCDD_CSOP_nmGetCan2TxErrorCount/1
  R_HALINCDD_CSOP_nmGetCan2RxErrorCount/1 -> [u8_pCan2RxErrorCount]
  R_HALINCDD_CSOP_nmGetCan2TxErrorCount/1 -> [u8_pCan2TxErrorCount]
  Constant13/1 -> R_HALINCDD_CSOP_nmGetCan2RxErrorCount/2
  Constant17/1 -> R_HALINCDD_CSOP_nmGetCan3TxErrorCount/2
  Constant18/1 -> R_HALINCDD_CSOP_nmGetCan3RxErrorCount/1
  Constant19/1 -> R_HALINCDD_CSOP_nmGetCan3TxErrorCount/1
  R_HALINCDD_CSOP_nmGetCan3RxErrorCount/1 -> [u8_pCan3RxErrorCount]
  R_HALINCDD_CSOP_nmGetCan3TxErrorCount/1 -> [u8_pCan3TxErrorCount]
  Constant20/1 -> R_HALINCDD_CSOP_nmGetCan3RxErrorCount/2
  Constant22/1 -> R_HALINCDD_CSOP_nmGetCan4RxErrorCount/1
  Constant24/1 -> R_HALINCDD_CSOP_nmGetCan4RxErrorCount/2
  Constant23/1 -> R_HALINCDD_CSOP_nmGetCan4TxErrorCount/1
  R_HALINCDD_CSOP_nmGetCan4TxErrorCount/1 -> [u8_pCan4TxErrorCount]
  Constant21/1 -> R_HALINCDD_CSOP_nmGetCan4TxErrorCount/2
  R_HALINCDD_CSOP_nmGetCan4RxErrorCount/1 -> [u8_pCan4RxErrorCount]
  Constant26/1 -> R_HALINCDD_CSOP_nmGetCan5RxErrorCount/1
  Constant28/1 -> R_HALINCDD_CSOP_nmGetCan5RxErrorCount/2
  Constant27/1 -> R_HALINCDD_CSOP_nmGetCan5TxErrorCount/1
  R_HALINCDD_CSOP_nmGetCan5TxErrorCount/1 -> [u8_pCan5TxErrorCount]
  Constant25/1 -> R_HALINCDD_CSOP_nmGetCan5TxErrorCount/2
  R_HALINCDD_CSOP_nmGetCan5RxErrorCount/1 -> [u8_pCan5RxErrorCount]
  Constant31/1 -> R_HALINCDD_CSOP_nmGetCan6TxErrorCount/1
  Constant32/1 -> R_HALINCDD_CSOP_nmGetCan6RxErrorCount/2
  Constant29/1 -> R_HALINCDD_CSOP_nmGetCan6TxErrorCount/2
  Constant30/1 -> R_HALINCDD_CSOP_nmGetCan6RxErrorCount/1
  R_HALINCDD_CSOP_nmGetCan6RxErrorCount/1 -> [u8_pCan6RxErrorCount]
  R_HALINCDD_CSOP_nmGetCan6TxErrorCount/1 -> [u8_pCan6TxErrorCount]
  [u8_pCan1RxErrorCount] -> Halin_CDD/88(VHAL_CAN1RxErrorCount_raw)
  [u8_pCan1TxErrorCount] -> Halin_CDD/89(VHAL_CAN1TxErrorCount_raw)
  [u8_pCan2RxErrorCount] -> Halin_CDD/90(VHAL_CAN2RxErrorCount_raw)
  [u8_pCan2TxErrorCount] -> Halin_CDD/91(VHAL_CAN2TxErrorCount_raw)
  [u8_pCan3RxErrorCount] -> Halin_CDD/92(VHAL_CAN3RxErrorCount_cnt)
  [u8_pCan3TxErrorCount] -> Halin_CDD/93(VHAL_CAN3TxErrorCount_raw)
  [u8_pCan4RxErrorCount] -> Halin_CDD/94(VHAL_CAN4RxErrorCount_raw)
  [u8_pCan4TxErrorCount] -> Halin_CDD/95(VHAL_CAN4TxErrorCount_raw)
  [u8_pCan5RxErrorCount] -> Halin_CDD/96(VHAL_CAN5RxErrorCount_raw)
  [u8_pCan5TxErrorCount] -> Halin_CDD/97(VHAL_CAN5TxErrorCount_raw)
  OUTP_AFTER/10(DTC_Constant_Array) -> [DTC_Constant_Array]
  [DTC_Constant_Array] -> R_UDSCDD_CSOP_SetDTCStatus/3(DTC_Constant_Array)
  [u8_pCan6RxErrorCount] -> Halin_CDD/98(VHAL_CAN6RxErrorCount_raw)
  [u8_pCan6TxErrorCount] -> Halin_CDD/99(VHAL_CAN6TxErrorCount_raw)
  hcu_main_sched/17(trig_SetDID()) -> [trig_SetDID]
  Ground6/1 -> HAL_IN/51
  Ground8/1 -> HAL_IN/53
  Ground7/1 -> HAL_IN/52
  R_CAN5_TBOX1_CAN5_SG_TBOX1_read/1 -> Terminator/1
  R_CAN5_TBOX2_CAN5_SG_TBOX2_read/1 -> Terminator6/1
  R_CAN5_TBOX3_CAN5_SG_TBOX3_read/1 -> Terminator7/1
  [trig_GetDID] -> DIDGet_Subsystem/Trigger
  DIDGet_Subsystem/1(BHAL_DID_outputs) -> [BHAL_DID_outputs]
  [BOUTP_DIDSetData_outputs] -> DIDSet_Subsystem/1(BOUTP_DIDSetData_outputs)
  [BHAL_DID_outputs] -> DIDSet_Subsystem/2(BHAL_DID_outputs)
  [trig_SetDID] -> DIDSet_Subsystem/Trigger
  [BINP_CAN1_outputs] -> Bus Creator/1  "BINP_CAN1_outputs"
  [BINP_CAN2_outputs] -> Bus Creator/2  "BINP_CAN2_outputs"
  [BINP_CAN3_outputs] -> Bus Creator/3  "BINP_CAN3_outputs"
  [BINP_CAN4_outputs] -> Bus Creator/4  "BINP_CAN4_outputs"
  [BINP_CAN5_outputs] -> Bus Creator/5  "BINP_CAN5_outputs"
  [BINP_CAN6_outputs] -> Bus Creator/6  "BINP_CAN6_outputs"
  Bus Creator/1 -> [BINP_CANx_outputs]
  [BINP_CANx_outputs] -> OUTP_AFTER/6(BINP_CANx_outputs)
  [BINP_APM_outputs] -> Bus Creator/7  "BINP_APM_outputs"
